simulink library "mbd_s32k1xx_ec_toolbox"  (Simulink 9.0)
settings: Solver=FixedStepDiscrete  StartTime=0.0  StopTime=10.0  FixedStep=0.1  RelTol=1e-3  EnableMultiTasking=on
InitFcn:
  | mbd_s32k_consistency_checks(bdroot(gcs));
(part 4 of 8)

== system mbd_s32k1xx_ec_toolbox/Core and System Blocks/DMA Blocks ==
  eDMA_Config : S-Function  FunctionName=edma_s32k_config  SFunctionDeploymentMode=off  EnableBusSupport=off  mask(edma_s32k_config){channel=0, show_advanced_tab=on, channel_advanced_checkbox=off, show_enabled=on, arbitration=EDMA_ARBITRATION_FIXED_PRIORITY, halt_on_error=false, channel0priority=EDMA_CHN_DEFAULT_PRIORITY, channel0requestsource=EDMA_REQ_DISABLED, channel0enable=off, channel1priority=EDMA_CHN_DEFAULT_PRIORITY, channel1requestsource=EDMA_REQ_DISABLED, channel1enable=off, channel2priority=EDMA_CHN_DEFAULT_PRIORITY, channel2requestsource=EDMA_REQ_DISABLED, channel2enable=off, channel3priority=EDMA_CHN_DEFAULT_PRIORITY, channel3requestsource=EDMA_REQ_DISABLED, channel3enable=off, channel4priority=EDMA_CHN_DEFAULT_PRIORITY, channel4requestsource=EDMA_REQ_DISABLED, channel4enable=off, channel5priority=EDMA_CHN_DEFAULT_PRIORITY, channel5requestsource=EDMA_REQ_DISABLED, channel5enable=off, channel6priority=EDMA_CHN_DEFAULT_PRIORITY, channel6requestsource=EDMA_REQ_DISABLED, channel6enable=off, channel7priority=EDMA_CHN_DEFAULT_PRIORITY, channel7requestsource=EDMA_REQ_DISABLED, channel7enable=off, channel8priority=EDMA_CHN_DEFAULT_PRIORITY, channel8requestsource=EDMA_REQ_DISABLED, channel8enable=off, channel9priority=EDMA_CHN_DEFAULT_PRIORITY, channel9requestsource=EDMA_REQ_DISABLED, channel9enable=off, channel10priority=EDMA_CHN_DEFAULT_PRIORITY, channel10requestsource=EDMA_REQ_DISABLED, channel10enable=off, channel11priority=EDMA_CHN_DEFAULT_PRIORITY, channel11requestsource=EDMA_REQ_DISABLED, channel11enable=off, channel12priority=EDMA_CHN_DEFAULT_PRIORITY, channel12requestsource=EDMA_REQ_DISABLED, channel12enable=off, channel13priority=EDMA_CHN_DEFAULT_PRIORITY, channel13requestsource=EDMA_REQ_DISABLED, channel13enable=off, channel14priority=EDMA_CHN_DEFAULT_PRIORITY, channel14requestsource=EDMA_REQ_DISABLED, channel14enable=off, channel15priority=EDMA_CHN_DEFAULT_PRIORITY, channel15requestsource=EDMA_REQ_DISABLED, channel15enable=off}
      mask prompts: show_advanced_tab "Show advanced global settings"; channel_advanced_checkbox "Show channel settings"; show_enabled "Show enabled channels"; halt_on_error "Halt on error"; channel0priority "Priority"; channel0requestsource "DMA request source"; channel0enable "Enable"; channel1priority "Priority"; channel1requestsource "DMA request source"; channel1enable "Enable"; channel2priority "Priority"; channel2requestsource "DMA request source"; channel2enable "Enable"; channel3priority "Priority"; channel3requestsource "DMA request source"; channel3enable "Enable"; channel4priority "Priority"; channel4requestsource "DMA request source"; channel4enable "Enable"; channel5priority "Priority"; channel5requestsource "DMA request source"; channel5enable "Enable"; channel6priority "Priority"; channel6requestsource "DMA request source"; channel6enable "Enable"; channel7priority "Priority"; channel7requestsource "DMA request source"; channel7enable "Enable"; channel8priority "Priority"; channel8requestsource "DMA request source"; channel8enable "Enable"; channel9priority "Priority"; channel9requestsource "DMA request source"; channel9enable "Enable"; channel10priority "Priority"; channel10requestsource "DMA request source"; channel10enable "Enable"; channel11priority "Priority"; channel11requestsource "DMA request source"; channel11enable "Enable"; channel12priority "Priority"; channel12requestsource "DMA request source"; channel12enable "Enable"; channel13priority "Priority"; channel13requestsource "DMA request source"; channel13enable "Enable"; channel14priority "Priority"; channel14requestsource "DMA request source"; channel14enable "Enable"; channel15priority "Priority"; channel15requestsource "DMA request source"; channel15enable "Enable"
      mask help: This block allows the user to configure the eDMA module and all of its channels.
      mask init:
      | maskStr = mbd_s32k_edma_config_init();
      settings: NameChangeFcn=mbd_s32k_name_check(gcb);
      mask Help: web(fullfile(mbd_s32k_block_help, 'edma', 'edma_config.html'));
      mask TypeOptions channel: 0 | 1 | 2 | 3 | 4 | 5 | 6 | 7 | 8 | 9 | 10 | 11 | 12 | 13 | 14 | 15
      mask Callback channel: mbd_s32k_edma_config_cbk()
      mask Callback show_advanced_tab: mbd_s32k_edma_config_cbk()
      mask Callback channel_advanced_checkbox: mbd_s32k_edma_config_cbk()
      mask Callback show_enabled: mbd_s32k_edma_config_en_chn()
      mask TypeOptions arbitration: EDMA_ARBITRATION_FIXED_PRIORITY | EDMA_ARBITRATION_ROUND_ROBIN
      mask TypeOptions halt_on_error: false | true
      mask TypeOptions channel0priority: EDMA_CHN_DEFAULT_PRIORITY | EDMA_CHN_PRIORITY_0 | EDMA_CHN_PRIORITY_1 | EDMA_CHN_PRIORITY_2 | EDMA_CHN_PRIORITY_3 | EDMA_CHN_PRIORITY_4 | EDMA_CHN_PRIORITY_5 | EDMA_CHN_PRIORITY_6 | EDMA_CHN_PRIORITY_7 | EDMA_CHN_PRIORITY_8 | EDMA_CHN_PRIORITY_9 | EDMA_CHN_PRIORITY_10 | EDMA_CHN_PRIORITY_11 | EDMA_CHN_PRIORITY_12 | EDMA_CHN_PRIORITY_13 | EDMA_CHN_PRIORITY_14 | EDMA_CHN_PRIORITY_15
      mask Callback channel0priority: mbd_s32k_edma_transfer_priority_cbk('0')
      mask TypeOptions channel0requestsource: EDMA_REQ_DISABLED | EDMA_REQ_LPUART0_RX | EDMA_REQ_LPUART0_TX | EDMA_REQ_LPUART1_RX | EDMA_REQ_LPUART1_TX | EDMA_REQ_FLEXIO_SHIFTER0 | EDMA_REQ_FLEXIO_SHIFTER1 | EDMA_REQ_FLEXIO_SHIFTER2 | EDMA_REQ_FLEXIO_SHIFTER3 | EDMA_REQ_LPSPI0_RX | EDMA_REQ_LPSPI0_TX | EDMA_REQ_LPSPI1_RX | EDMA_REQ_LPSPI1_TX | EDMA_REQ_FTM1_CHANNEL_0 | EDMA_REQ_FTM1_CHANNEL_1 | EDMA_REQ_FTM1_CHANNEL_2 | EDMA_REQ_FTM1_CHANNEL_3 | EDMA_REQ_FTM1_CHANNEL_4 | EDMA_REQ_FTM1_CHANNEL_5 | EDMA_REQ_FTM1_CHANNEL_6 | EDMA_REQ_FTM1_CHANNEL_7 | EDMA_REQ_FTM2_CHANNEL_0 | EDMA_REQ_FTM2_CHANNEL_1 | EDMA_REQ_FTM2_CHANNEL_2 | EDMA_REQ_FTM2_CHANNEL_3 | EDMA_REQ_FTM2_CHANNEL_4 | EDMA_REQ_FTM2_CHANNEL_5 | EDMA_REQ_FTM2_CHANNEL_6 | EDMA_REQ_FTM2_CHANNEL_7 | EDMA_REQ_FTM0_OR_CH0_CH7 | EDMA_REQ_FTM3_OR_CH0_CH7 | EDMA_REQ_ADC0 | EDMA_REQ_ADC1 | EDMA_REQ_LPI2C0_RX | EDMA_REQ_LPI2C0_TX | EDMA_REQ_PDB0 | EDMA_REQ_PDB1 | EDMA_REQ_CMP0 | EDMA_REQ_PORTA | EDMA_REQ_PORTB | EDMA_REQ_PORTC | EDMA_REQ_PORTD | EDMA_REQ_PORTE | EDMA_REQ_FLEXCAN0 | EDMA_REQ_FLEXCAN1 | EDMA_REQ_LPTMR0 | EDMA_REQ_DMAMUX_ALWAYS_ENABLED0 | EDMA_REQ_DMAMUX_ALWAYS_ENABLED1
      mask Callback channel0enable: mbd_s32k_edma_config_en_chn()
      mask TypeOptions channel1priority: EDMA_CHN_DEFAULT_PRIORITY | EDMA_CHN_PRIORITY_0 | EDMA_CHN_PRIORITY_1 | EDMA_CHN_PRIORITY_2 | EDMA_CHN_PRIORITY_3 | EDMA_CHN_PRIORITY_4 | EDMA_CHN_PRIORITY_5 | EDMA_CHN_PRIORITY_6 | EDMA_CHN_PRIORITY_7 | EDMA_CHN_PRIORITY_8 | EDMA_CHN_PRIORITY_9 | EDMA_CHN_PRIORITY_10 | EDMA_CHN_PRIORITY_11 | EDMA_CHN_PRIORITY_12 | EDMA_CHN_PRIORITY_13 | EDMA_CHN_PRIORITY_14 | EDMA_CHN_PRIORITY_15
      mask Callback channel1priority: mbd_s32k_edma_transfer_priority_cbk('1')
      mask TypeOptions channel1requestsource: EDMA_REQ_DISABLED | EDMA_REQ_LPUART0_RX | EDMA_REQ_LPUART0_TX | EDMA_REQ_LPUART1_RX | EDMA_REQ_LPUART1_TX | EDMA_REQ_FLEXIO_SHIFTER0 | EDMA_REQ_FLEXIO_SHIFTER1 | EDMA_REQ_FLEXIO_SHIFTER2 | EDMA_REQ_FLEXIO_SHIFTER3 | EDMA_REQ_LPSPI0_RX | EDMA_REQ_LPSPI0_TX | EDMA_REQ_LPSPI1_RX | EDMA_REQ_LPSPI1_TX | EDMA_REQ_FTM1_CHANNEL_0 | EDMA_REQ_FTM1_CHANNEL_1 | EDMA_REQ_FTM1_CHANNEL_2 | EDMA_REQ_FTM1_CHANNEL_3 | EDMA_REQ_FTM1_CHANNEL_4 | EDMA_REQ_FTM1_CHANNEL_5 | EDMA_REQ_FTM1_CHANNEL_6 | EDMA_REQ_FTM1_CHANNEL_7 | EDMA_REQ_FTM2_CHANNEL_0 | EDMA_REQ_FTM2_CHANNEL_1 | EDMA_REQ_FTM2_CHANNEL_2 | EDMA_REQ_FTM2_CHANNEL_3 | EDMA_REQ_FTM2_CHANNEL_4 | EDMA_REQ_FTM2_CHANNEL_5 | EDMA_REQ_FTM2_CHANNEL_6 | EDMA_REQ_FTM2_CHANNEL_7 | EDMA_REQ_FTM0_OR_CH0_CH7 | EDMA_REQ_FTM3_OR_CH0_CH7 | EDMA_REQ_ADC0 | EDMA_REQ_ADC1 | EDMA_REQ_LPI2C0_RX | EDMA_REQ_LPI2C0_TX | EDMA_REQ_PDB0 | EDMA_REQ_PDB1 | EDMA_REQ_CMP0 | EDMA_REQ_PORTA | EDMA_REQ_PORTB | EDMA_REQ_PORTC | EDMA_REQ_PORTD | EDMA_REQ_PORTE | EDMA_REQ_FLEXCAN0 | EDMA_REQ_FLEXCAN1 | EDMA_REQ_LPTMR0 | EDMA_REQ_DMAMUX_ALWAYS_ENABLED0 | EDMA_REQ_DMAMUX_ALWAYS_ENABLED1
      mask Callback channel1enable: mbd_s32k_edma_config_en_chn()
      mask TypeOptions channel2priority: EDMA_CHN_DEFAULT_PRIORITY | EDMA_CHN_PRIORITY_0 | EDMA_CHN_PRIORITY_1 | EDMA_CHN_PRIORITY_2 | EDMA_CHN_PRIORITY_3 | EDMA_CHN_PRIORITY_4 | EDMA_CHN_PRIORITY_5 | EDMA_CHN_PRIORITY_6 | EDMA_CHN_PRIORITY_7 | EDMA_CHN_PRIORITY_8 | EDMA_CHN_PRIORITY_9 | EDMA_CHN_PRIORITY_10 | EDMA_CHN_PRIORITY_11 | EDMA_CHN_PRIORITY_12 | EDMA_CHN_PRIORITY_13 | EDMA_CHN_PRIORITY_14 | EDMA_CHN_PRIORITY_15
      mask Callback channel2priority: mbd_s32k_edma_transfer_priority_cbk('2')
      mask TypeOptions channel2requestsource: EDMA_REQ_DISABLED | EDMA_REQ_LPUART0_RX | EDMA_REQ_LPUART0_TX | EDMA_REQ_LPUART1_RX | EDMA_REQ_LPUART1_TX | EDMA_REQ_FLEXIO_SHIFTER0 | EDMA_REQ_FLEXIO_SHIFTER1 | EDMA_REQ_FLEXIO_SHIFTER2 | EDMA_REQ_FLEXIO_SHIFTER3 | EDMA_REQ_LPSPI0_RX | EDMA_REQ_LPSPI0_TX | EDMA_REQ_LPSPI1_RX | EDMA_REQ_LPSPI1_TX | EDMA_REQ_FTM1_CHANNEL_0 | EDMA_REQ_FTM1_CHANNEL_1 | EDMA_REQ_FTM1_CHANNEL_2 | EDMA_REQ_FTM1_CHANNEL_3 | EDMA_REQ_FTM1_CHANNEL_4 | EDMA_REQ_FTM1_CHANNEL_5 | EDMA_REQ_FTM1_CHANNEL_6 | EDMA_REQ_FTM1_CHANNEL_7 | EDMA_REQ_FTM2_CHANNEL_0 | EDMA_REQ_FTM2_CHANNEL_1 | EDMA_REQ_FTM2_CHANNEL_2 | EDMA_REQ_FTM2_CHANNEL_3 | EDMA_REQ_FTM2_CHANNEL_4 | EDMA_REQ_FTM2_CHANNEL_5 | EDMA_REQ_FTM2_CHANNEL_6 | EDMA_REQ_FTM2_CHANNEL_7 | EDMA_REQ_FTM0_OR_CH0_CH7 | EDMA_REQ_FTM3_OR_CH0_CH7 | EDMA_REQ_ADC0 | EDMA_REQ_ADC1 | EDMA_REQ_LPI2C0_RX | EDMA_REQ_LPI2C0_TX | EDMA_REQ_PDB0 | EDMA_REQ_PDB1 | EDMA_REQ_CMP0 | EDMA_REQ_PORTA | EDMA_REQ_PORTB | EDMA_REQ_PORTC | EDMA_REQ_PORTD | EDMA_REQ_PORTE | EDMA_REQ_FLEXCAN0 | EDMA_REQ_FLEXCAN1 | EDMA_REQ_LPTMR0 | EDMA_REQ_DMAMUX_ALWAYS_ENABLED0 | EDMA_REQ_DMAMUX_ALWAYS_ENABLED1
      mask Callback channel2enable: mbd_s32k_edma_config_en_chn()
      mask TypeOptions channel3priority: EDMA_CHN_DEFAULT_PRIORITY | EDMA_CHN_PRIORITY_0 | EDMA_CHN_PRIORITY_1 | EDMA_CHN_PRIORITY_2 | EDMA_CHN_PRIORITY_3 | EDMA_CHN_PRIORITY_4 | EDMA_CHN_PRIORITY_5 | EDMA_CHN_PRIORITY_6 | EDMA_CHN_PRIORITY_7 | EDMA_CHN_PRIORITY_8 | EDMA_CHN_PRIORITY_9 | EDMA_CHN_PRIORITY_10 | EDMA_CHN_PRIORITY_11 | EDMA_CHN_PRIORITY_12 | EDMA_CHN_PRIORITY_13 | EDMA_CHN_PRIORITY_14 | EDMA_CHN_PRIORITY_15
      mask Callback channel3priority: mbd_s32k_edma_transfer_priority_cbk('3')
      mask TypeOptions channel3requestsource: EDMA_REQ_DISABLED | EDMA_REQ_LPUART0_RX | EDMA_REQ_LPUART0_TX | EDMA_REQ_LPUART1_RX | EDMA_REQ_LPUART1_TX | EDMA_REQ_FLEXIO_SHIFTER0 | EDMA_REQ_FLEXIO_SHIFTER1 | EDMA_REQ_FLEXIO_SHIFTER2 | EDMA_REQ_FLEXIO_SHIFTER3 | EDMA_REQ_LPSPI0_RX | EDMA_REQ_LPSPI0_TX | EDMA_REQ_LPSPI1_RX | EDMA_REQ_LPSPI1_TX | EDMA_REQ_FTM1_CHANNEL_0 | EDMA_REQ_FTM1_CHANNEL_1 | EDMA_REQ_FTM1_CHANNEL_2 | EDMA_REQ_FTM1_CHANNEL_3 | EDMA_REQ_FTM1_CHANNEL_4 | EDMA_REQ_FTM1_CHANNEL_5 | EDMA_REQ_FTM1_CHANNEL_6 | EDMA_REQ_FTM1_CHANNEL_7 | EDMA_REQ_FTM2_CHANNEL_0 | EDMA_REQ_FTM2_CHANNEL_1 | EDMA_REQ_FTM2_CHANNEL_2 | EDMA_REQ_FTM2_CHANNEL_3 | EDMA_REQ_FTM2_CHANNEL_4 | EDMA_REQ_FTM2_CHANNEL_5 | EDMA_REQ_FTM2_CHANNEL_6 | EDMA_REQ_FTM2_CHANNEL_7 | EDMA_REQ_FTM0_OR_CH0_CH7 | EDMA_REQ_FTM3_OR_CH0_CH7 | EDMA_REQ_ADC0 | EDMA_REQ_ADC1 | EDMA_REQ_LPI2C0_RX | EDMA_REQ_LPI2C0_TX | EDMA_REQ_PDB0 | EDMA_REQ_PDB1 | EDMA_REQ_CMP0 | EDMA_REQ_PORTA | EDMA_REQ_PORTB | EDMA_REQ_PORTC | EDMA_REQ_PORTD | EDMA_REQ_PORTE | EDMA_REQ_FLEXCAN0 | EDMA_REQ_FLEXCAN1 | EDMA_REQ_LPTMR0 | EDMA_REQ_DMAMUX_ALWAYS_ENABLED0 | EDMA_REQ_DMAMUX_ALWAYS_ENABLED1
      mask Callback channel3enable: mbd_s32k_edma_config_en_chn()
      mask TypeOptions channel4priority: EDMA_CHN_DEFAULT_PRIORITY | EDMA_CHN_PRIORITY_0 | EDMA_CHN_PRIORITY_1 | EDMA_CHN_PRIORITY_2 | EDMA_CHN_PRIORITY_3 | EDMA_CHN_PRIORITY_4 | EDMA_CHN_PRIORITY_5 | EDMA_CHN_PRIORITY_6 | EDMA_CHN_PRIORITY_7 | EDMA_CHN_PRIORITY_8 | EDMA_CHN_PRIORITY_9 | EDMA_CHN_PRIORITY_10 | EDMA_CHN_PRIORITY_11 | EDMA_CHN_PRIORITY_12 | EDMA_CHN_PRIORITY_13 | EDMA_CHN_PRIORITY_14 | EDMA_CHN_PRIORITY_15
      mask Callback channel4priority: mbd_s32k_edma_transfer_priority_cbk('4')
      mask TypeOptions channel4requestsource: EDMA_REQ_DISABLED | EDMA_REQ_LPUART0_RX | EDMA_REQ_LPUART0_TX | EDMA_REQ_LPUART1_RX | EDMA_REQ_LPUART1_TX | EDMA_REQ_FLEXIO_SHIFTER0 | EDMA_REQ_FLEXIO_SHIFTER1 | EDMA_REQ_FLEXIO_SHIFTER2 | EDMA_REQ_FLEXIO_SHIFTER3 | EDMA_REQ_LPSPI0_RX | EDMA_REQ_LPSPI0_TX | EDMA_REQ_LPSPI1_RX | EDMA_REQ_LPSPI1_TX | EDMA_REQ_FTM1_CHANNEL_0 | EDMA_REQ_FTM1_CHANNEL_1 | EDMA_REQ_FTM1_CHANNEL_2 | EDMA_REQ_FTM1_CHANNEL_3 | EDMA_REQ_FTM1_CHANNEL_4 | EDMA_REQ_FTM1_CHANNEL_5 | EDMA_REQ_FTM1_CHANNEL_6 | EDMA_REQ_FTM1_CHANNEL_7 | EDMA_REQ_FTM2_CHANNEL_0 | EDMA_REQ_FTM2_CHANNEL_1 | EDMA_REQ_FTM2_CHANNEL_2 | EDMA_REQ_FTM2_CHANNEL_3 | EDMA_REQ_FTM2_CHANNEL_4 | EDMA_REQ_FTM2_CHANNEL_5 | EDMA_REQ_FTM2_CHANNEL_6 | EDMA_REQ_FTM2_CHANNEL_7 | EDMA_REQ_FTM0_OR_CH0_CH7 | EDMA_REQ_FTM3_OR_CH0_CH7 | EDMA_REQ_ADC0 | EDMA_REQ_ADC1 | EDMA_REQ_LPI2C0_RX | EDMA_REQ_LPI2C0_TX | EDMA_REQ_PDB0 | EDMA_REQ_PDB1 | EDMA_REQ_CMP0 | EDMA_REQ_PORTA | EDMA_REQ_PORTB | EDMA_REQ_PORTC | EDMA_REQ_PORTD | EDMA_REQ_PORTE | EDMA_REQ_FLEXCAN0 | EDMA_REQ_FLEXCAN1 | EDMA_REQ_LPTMR0 | EDMA_REQ_DMAMUX_ALWAYS_ENABLED0 | EDMA_REQ_DMAMUX_ALWAYS_ENABLED1
      mask Callback channel4enable: mbd_s32k_edma_config_en_chn()
      mask TypeOptions channel5priority: EDMA_CHN_DEFAULT_PRIORITY | EDMA_CHN_PRIORITY_0 | EDMA_CHN_PRIORITY_1 | EDMA_CHN_PRIORITY_2 | EDMA_CHN_PRIORITY_3 | EDMA_CHN_PRIORITY_4 | EDMA_CHN_PRIORITY_5 | EDMA_CHN_PRIORITY_6 | EDMA_CHN_PRIORITY_7 | EDMA_CHN_PRIORITY_8 | EDMA_CHN_PRIORITY_9 | EDMA_CHN_PRIORITY_10 | EDMA_CHN_PRIORITY_11 | EDMA_CHN_PRIORITY_12 | EDMA_CHN_PRIORITY_13 | EDMA_CHN_PRIORITY_14 | EDMA_CHN_PRIORITY_15
      mask Callback channel5priority: mbd_s32k_edma_transfer_priority_cbk('5')
      mask TypeOptions channel5requestsource: EDMA_REQ_DISABLED | EDMA_REQ_LPUART0_RX | EDMA_REQ_LPUART0_TX | EDMA_REQ_LPUART1_RX | EDMA_REQ_LPUART1_TX | EDMA_REQ_FLEXIO_SHIFTER0 | EDMA_REQ_FLEXIO_SHIFTER1 | EDMA_REQ_FLEXIO_SHIFTER2 | EDMA_REQ_FLEXIO_SHIFTER3 | EDMA_REQ_LPSPI0_RX | EDMA_REQ_LPSPI0_TX | EDMA_REQ_LPSPI1_RX | EDMA_REQ_LPSPI1_TX | EDMA_REQ_FTM1_CHANNEL_0 | EDMA_REQ_FTM1_CHANNEL_1 | EDMA_REQ_FTM1_CHANNEL_2 | EDMA_REQ_FTM1_CHANNEL_3 | EDMA_REQ_FTM1_CHANNEL_4 | EDMA_REQ_FTM1_CHANNEL_5 | EDMA_REQ_FTM1_CHANNEL_6 | EDMA_REQ_FTM1_CHANNEL_7 | EDMA_REQ_FTM2_CHANNEL_0 | EDMA_REQ_FTM2_CHANNEL_1 | EDMA_REQ_FTM2_CHANNEL_2 | EDMA_REQ_FTM2_CHANNEL_3 | EDMA_REQ_FTM2_CHANNEL_4 | EDMA_REQ_FTM2_CHANNEL_5 | EDMA_REQ_FTM2_CHANNEL_6 | EDMA_REQ_FTM2_CHANNEL_7 | EDMA_REQ_FTM0_OR_CH0_CH7 | EDMA_REQ_FTM3_OR_CH0_CH7 | EDMA_REQ_ADC0 | EDMA_REQ_ADC1 | EDMA_REQ_LPI2C0_RX | EDMA_REQ_LPI2C0_TX | EDMA_REQ_PDB0 | EDMA_REQ_PDB1 | EDMA_REQ_CMP0 | EDMA_REQ_PORTA | EDMA_REQ_PORTB | EDMA_REQ_PORTC | EDMA_REQ_PORTD | EDMA_REQ_PORTE | EDMA_REQ_FLEXCAN0 | EDMA_REQ_FLEXCAN1 | EDMA_REQ_LPTMR0 | EDMA_REQ_DMAMUX_ALWAYS_ENABLED0 | EDMA_REQ_DMAMUX_ALWAYS_ENABLED1
      mask Callback channel5enable: mbd_s32k_edma_config_en_chn()
      mask TypeOptions channel6priority: EDMA_CHN_DEFAULT_PRIORITY | EDMA_CHN_PRIORITY_0 | EDMA_CHN_PRIORITY_1 | EDMA_CHN_PRIORITY_2 | EDMA_CHN_PRIORITY_3 | EDMA_CHN_PRIORITY_4 | EDMA_CHN_PRIORITY_5 | EDMA_CHN_PRIORITY_6 | EDMA_CHN_PRIORITY_7 | EDMA_CHN_PRIORITY_8 | EDMA_CHN_PRIORITY_9 | EDMA_CHN_PRIORITY_10 | EDMA_CHN_PRIORITY_11 | EDMA_CHN_PRIORITY_12 | EDMA_CHN_PRIORITY_13 | EDMA_CHN_PRIORITY_14 | EDMA_CHN_PRIORITY_15
      mask Callback channel6priority: mbd_s32k_edma_transfer_priority_cbk('6')
      mask TypeOptions channel6requestsource: EDMA_REQ_DISABLED | EDMA_REQ_LPUART0_RX | EDMA_REQ_LPUART0_TX | EDMA_REQ_LPUART1_RX | EDMA_REQ_LPUART1_TX | EDMA_REQ_FLEXIO_SHIFTER0 | EDMA_REQ_FLEXIO_SHIFTER1 | EDMA_REQ_FLEXIO_SHIFTER2 | EDMA_REQ_FLEXIO_SHIFTER3 | EDMA_REQ_LPSPI0_RX | EDMA_REQ_LPSPI0_TX | EDMA_REQ_LPSPI1_RX | EDMA_REQ_LPSPI1_TX | EDMA_REQ_FTM1_CHANNEL_0 | EDMA_REQ_FTM1_CHANNEL_1 | EDMA_REQ_FTM1_CHANNEL_2 | EDMA_REQ_FTM1_CHANNEL_3 | EDMA_REQ_FTM1_CHANNEL_4 | EDMA_REQ_FTM1_CHANNEL_5 | EDMA_REQ_FTM1_CHANNEL_6 | EDMA_REQ_FTM1_CHANNEL_7 | EDMA_REQ_FTM2_CHANNEL_0 | EDMA_REQ_FTM2_CHANNEL_1 | EDMA_REQ_FTM2_CHANNEL_2 | EDMA_REQ_FTM2_CHANNEL_3 | EDMA_REQ_FTM2_CHANNEL_4 | EDMA_REQ_FTM2_CHANNEL_5 | EDMA_REQ_FTM2_CHANNEL_6 | EDMA_REQ_FTM2_CHANNEL_7 | EDMA_REQ_FTM0_OR_CH0_CH7 | EDMA_REQ_FTM3_OR_CH0_CH7 | EDMA_REQ_ADC0 | EDMA_REQ_ADC1 | EDMA_REQ_LPI2C0_RX | EDMA_REQ_LPI2C0_TX | EDMA_REQ_PDB0 | EDMA_REQ_PDB1 | EDMA_REQ_CMP0 | EDMA_REQ_PORTA | EDMA_REQ_PORTB | EDMA_REQ_PORTC | EDMA_REQ_PORTD | EDMA_REQ_PORTE | EDMA_REQ_FLEXCAN0 | EDMA_REQ_FLEXCAN1 | EDMA_REQ_LPTMR0 | EDMA_REQ_DMAMUX_ALWAYS_ENABLED0 | EDMA_REQ_DMAMUX_ALWAYS_ENABLED1
      mask Callback channel6enable: mbd_s32k_edma_config_en_chn()
      mask TypeOptions channel7priority: EDMA_CHN_DEFAULT_PRIORITY | EDMA_CHN_PRIORITY_0 | EDMA_CHN_PRIORITY_1 | EDMA_CHN_PRIORITY_2 | EDMA_CHN_PRIORITY_3 | EDMA_CHN_PRIORITY_4 | EDMA_CHN_PRIORITY_5 | EDMA_CHN_PRIORITY_6 | EDMA_CHN_PRIORITY_7 | EDMA_CHN_PRIORITY_8 | EDMA_CHN_PRIORITY_9 | EDMA_CHN_PRIORITY_10 | EDMA_CHN_PRIORITY_11 | EDMA_CHN_PRIORITY_12 | EDMA_CHN_PRIORITY_13 | EDMA_CHN_PRIORITY_14 | EDMA_CHN_PRIORITY_15
      mask Callback channel7priority: mbd_s32k_edma_transfer_priority_cbk('7')
      mask TypeOptions channel7requestsource: EDMA_REQ_DISABLED | EDMA_REQ_LPUART0_RX | EDMA_REQ_LPUART0_TX | EDMA_REQ_LPUART1_RX | EDMA_REQ_LPUART1_TX | EDMA_REQ_FLEXIO_SHIFTER0 | EDMA_REQ_FLEXIO_SHIFTER1 | EDMA_REQ_FLEXIO_SHIFTER2 | EDMA_REQ_FLEXIO_SHIFTER3 | EDMA_REQ_LPSPI0_RX | EDMA_REQ_LPSPI0_TX | EDMA_REQ_LPSPI1_RX | EDMA_REQ_LPSPI1_TX | EDMA_REQ_FTM1_CHANNEL_0 | EDMA_REQ_FTM1_CHANNEL_1 | EDMA_REQ_FTM1_CHANNEL_2 | EDMA_REQ_FTM1_CHANNEL_3 | EDMA_REQ_FTM1_CHANNEL_4 | EDMA_REQ_FTM1_CHANNEL_5 | EDMA_REQ_FTM1_CHANNEL_6 | EDMA_REQ_FTM1_CHANNEL_7 | EDMA_REQ_FTM2_CHANNEL_0 | EDMA_REQ_FTM2_CHANNEL_1 | EDMA_REQ_FTM2_CHANNEL_2 | EDMA_REQ_FTM2_CHANNEL_3 | EDMA_REQ_FTM2_CHANNEL_4 | EDMA_REQ_FTM2_CHANNEL_5 | EDMA_REQ_FTM2_CHANNEL_6 | EDMA_REQ_FTM2_CHANNEL_7 | EDMA_REQ_FTM0_OR_CH0_CH7 | EDMA_REQ_FTM3_OR_CH0_CH7 | EDMA_REQ_ADC0 | EDMA_REQ_ADC1 | EDMA_REQ_LPI2C0_RX | EDMA_REQ_LPI2C0_TX | EDMA_REQ_PDB0 | EDMA_REQ_PDB1 | EDMA_REQ_CMP0 | EDMA_REQ_PORTA | EDMA_REQ_PORTB | EDMA_REQ_PORTC | EDMA_REQ_PORTD | EDMA_REQ_PORTE | EDMA_REQ_FLEXCAN0 | EDMA_REQ_FLEXCAN1 | EDMA_REQ_LPTMR0 | EDMA_REQ_DMAMUX_ALWAYS_ENABLED0 | EDMA_REQ_DMAMUX_ALWAYS_ENABLED1
      mask Callback channel7enable: mbd_s32k_edma_config_en_chn()
      mask TypeOptions channel8priority: EDMA_CHN_DEFAULT_PRIORITY | EDMA_CHN_PRIORITY_0 | EDMA_CHN_PRIORITY_1 | EDMA_CHN_PRIORITY_2 | EDMA_CHN_PRIORITY_3 | EDMA_CHN_PRIORITY_4 | EDMA_CHN_PRIORITY_5 | EDMA_CHN_PRIORITY_6 | EDMA_CHN_PRIORITY_7 | EDMA_CHN_PRIORITY_8 | EDMA_CHN_PRIORITY_9 | EDMA_CHN_PRIORITY_10 | EDMA_CHN_PRIORITY_11 | EDMA_CHN_PRIORITY_12 | EDMA_CHN_PRIORITY_13 | EDMA_CHN_PRIORITY_14 | EDMA_CHN_PRIORITY_15
      mask Callback channel8priority: mbd_s32k_edma_transfer_priority_cbk('8')
      mask TypeOptions channel8requestsource: EDMA_REQ_DISABLED | EDMA_REQ_LPUART0_RX | EDMA_REQ_LPUART0_TX | EDMA_REQ_LPUART1_RX | EDMA_REQ_LPUART1_TX | EDMA_REQ_FLEXIO_SHIFTER0 | EDMA_REQ_FLEXIO_SHIFTER1 | EDMA_REQ_FLEXIO_SHIFTER2 | EDMA_REQ_FLEXIO_SHIFTER3 | EDMA_REQ_LPSPI0_RX | EDMA_REQ_LPSPI0_TX | EDMA_REQ_LPSPI1_RX | EDMA_REQ_LPSPI1_TX | EDMA_REQ_FTM1_CHANNEL_0 | EDMA_REQ_FTM1_CHANNEL_1 | EDMA_REQ_FTM1_CHANNEL_2 | EDMA_REQ_FTM1_CHANNEL_3 | EDMA_REQ_FTM1_CHANNEL_4 | EDMA_REQ_FTM1_CHANNEL_5 | EDMA_REQ_FTM1_CHANNEL_6 | EDMA_REQ_FTM1_CHANNEL_7 | EDMA_REQ_FTM2_CHANNEL_0 | EDMA_REQ_FTM2_CHANNEL_1 | EDMA_REQ_FTM2_CHANNEL_2 | EDMA_REQ_FTM2_CHANNEL_3 | EDMA_REQ_FTM2_CHANNEL_4 | EDMA_REQ_FTM2_CHANNEL_5 | EDMA_REQ_FTM2_CHANNEL_6 | EDMA_REQ_FTM2_CHANNEL_7 | EDMA_REQ_FTM0_OR_CH0_CH7 | EDMA_REQ_FTM3_OR_CH0_CH7 | EDMA_REQ_ADC0 | EDMA_REQ_ADC1 | EDMA_REQ_LPI2C0_RX | EDMA_REQ_LPI2C0_TX | EDMA_REQ_PDB0 | EDMA_REQ_PDB1 | EDMA_REQ_CMP0 | EDMA_REQ_PORTA | EDMA_REQ_PORTB | EDMA_REQ_PORTC | EDMA_REQ_PORTD | EDMA_REQ_PORTE | EDMA_REQ_FLEXCAN0 | EDMA_REQ_FLEXCAN1 | EDMA_REQ_LPTMR0 | EDMA_REQ_DMAMUX_ALWAYS_ENABLED0 | EDMA_REQ_DMAMUX_ALWAYS_ENABLED1
      mask Callback channel8enable: mbd_s32k_edma_config_en_chn()
      mask TypeOptions channel9priority: EDMA_CHN_DEFAULT_PRIORITY | EDMA_CHN_PRIORITY_0 | EDMA_CHN_PRIORITY_1 | EDMA_CHN_PRIORITY_2 | EDMA_CHN_PRIORITY_3 | EDMA_CHN_PRIORITY_4 | EDMA_CHN_PRIORITY_5 | EDMA_CHN_PRIORITY_6 | EDMA_CHN_PRIORITY_7 | EDMA_CHN_PRIORITY_8 | EDMA_CHN_PRIORITY_9 | EDMA_CHN_PRIORITY_10 | EDMA_CHN_PRIORITY_11 | EDMA_CHN_PRIORITY_12 | EDMA_CHN_PRIORITY_13 | EDMA_CHN_PRIORITY_14 | EDMA_CHN_PRIORITY_15
      mask Callback channel9priority: mbd_s32k_edma_transfer_priority_cbk('9')
      mask TypeOptions channel9requestsource: EDMA_REQ_DISABLED | EDMA_REQ_LPUART0_RX | EDMA_REQ_LPUART0_TX | EDMA_REQ_LPUART1_RX | EDMA_REQ_LPUART1_TX | EDMA_REQ_FLEXIO_SHIFTER0 | EDMA_REQ_FLEXIO_SHIFTER1 | EDMA_REQ_FLEXIO_SHIFTER2 | EDMA_REQ_FLEXIO_SHIFTER3 | EDMA_REQ_LPSPI0_RX | EDMA_REQ_LPSPI0_TX | EDMA_REQ_LPSPI1_RX | EDMA_REQ_LPSPI1_TX | EDMA_REQ_FTM1_CHANNEL_0 | EDMA_REQ_FTM1_CHANNEL_1 | EDMA_REQ_FTM1_CHANNEL_2 | EDMA_REQ_FTM1_CHANNEL_3 | EDMA_REQ_FTM1_CHANNEL_4 | EDMA_REQ_FTM1_CHANNEL_5 | EDMA_REQ_FTM1_CHANNEL_6 | EDMA_REQ_FTM1_CHANNEL_7 | EDMA_REQ_FTM2_CHANNEL_0 | EDMA_REQ_FTM2_CHANNEL_1 | EDMA_REQ_FTM2_CHANNEL_2 | EDMA_REQ_FTM2_CHANNEL_3 | EDMA_REQ_FTM2_CHANNEL_4 | EDMA_REQ_FTM2_CHANNEL_5 | EDMA_REQ_FTM2_CHANNEL_6 | EDMA_REQ_FTM2_CHANNEL_7 | EDMA_REQ_FTM0_OR_CH0_CH7 | EDMA_REQ_FTM3_OR_CH0_CH7 | EDMA_REQ_ADC0 | EDMA_REQ_ADC1 | EDMA_REQ_LPI2C0_RX | EDMA_REQ_LPI2C0_TX | EDMA_REQ_PDB0 | EDMA_REQ_PDB1 | EDMA_REQ_CMP0 | EDMA_REQ_PORTA | EDMA_REQ_PORTB | EDMA_REQ_PORTC | EDMA_REQ_PORTD | EDMA_REQ_PORTE | EDMA_REQ_FLEXCAN0 | EDMA_REQ_FLEXCAN1 | EDMA_REQ_LPTMR0 | EDMA_REQ_DMAMUX_ALWAYS_ENABLED0 | EDMA_REQ_DMAMUX_ALWAYS_ENABLED1
      mask Callback channel9enable: mbd_s32k_edma_config_en_chn()
      mask TypeOptions channel10priority: EDMA_CHN_DEFAULT_PRIORITY | EDMA_CHN_PRIORITY_0 | EDMA_CHN_PRIORITY_1 | EDMA_CHN_PRIORITY_2 | EDMA_CHN_PRIORITY_3 | EDMA_CHN_PRIORITY_4 | EDMA_CHN_PRIORITY_5 | EDMA_CHN_PRIORITY_6 | EDMA_CHN_PRIORITY_7 | EDMA_CHN_PRIORITY_8 | EDMA_CHN_PRIORITY_9 | EDMA_CHN_PRIORITY_10 | EDMA_CHN_PRIORITY_11 | EDMA_CHN_PRIORITY_12 | EDMA_CHN_PRIORITY_13 | EDMA_CHN_PRIORITY_14 | EDMA_CHN_PRIORITY_15
      mask Callback channel10priority: mbd_s32k_edma_transfer_priority_cbk('10')
      mask TypeOptions channel10requestsource: EDMA_REQ_DISABLED | EDMA_REQ_LPUART0_RX | EDMA_REQ_LPUART0_TX | EDMA_REQ_LPUART1_RX | EDMA_REQ_LPUART1_TX | EDMA_REQ_FLEXIO_SHIFTER0 | EDMA_REQ_FLEXIO_SHIFTER1 | EDMA_REQ_FLEXIO_SHIFTER2 | EDMA_REQ_FLEXIO_SHIFTER3 | EDMA_REQ_LPSPI0_RX | EDMA_REQ_LPSPI0_TX | EDMA_REQ_LPSPI1_RX | EDMA_REQ_LPSPI1_TX | EDMA_REQ_FTM1_CHANNEL_0 | EDMA_REQ_FTM1_CHANNEL_1 | EDMA_REQ_FTM1_CHANNEL_2 | EDMA_REQ_FTM1_CHANNEL_3 | EDMA_REQ_FTM1_CHANNEL_4 | EDMA_REQ_FTM1_CHANNEL_5 | EDMA_REQ_FTM1_CHANNEL_6 | EDMA_REQ_FTM1_CHANNEL_7 | EDMA_REQ_FTM2_CHANNEL_0 | EDMA_REQ_FTM2_CHANNEL_1 | EDMA_REQ_FTM2_CHANNEL_2 | EDMA_REQ_FTM2_CHANNEL_3 | EDMA_REQ_FTM2_CHANNEL_4 | EDMA_REQ_FTM2_CHANNEL_5 | EDMA_REQ_FTM2_CHANNEL_6 | EDMA_REQ_FTM2_CHANNEL_7 | EDMA_REQ_FTM0_OR_CH0_CH7 | EDMA_REQ_FTM3_OR_CH0_CH7 | EDMA_REQ_ADC0 | EDMA_REQ_ADC1 | EDMA_REQ_LPI2C0_RX | EDMA_REQ_LPI2C0_TX | EDMA_REQ_PDB0 | EDMA_REQ_PDB1 | EDMA_REQ_CMP0 | EDMA_REQ_PORTA | EDMA_REQ_PORTB | EDMA_REQ_PORTC | EDMA_REQ_PORTD | EDMA_REQ_PORTE | EDMA_REQ_FLEXCAN0 | EDMA_REQ_FLEXCAN1 | EDMA_REQ_LPTMR0 | EDMA_REQ_DMAMUX_ALWAYS_ENABLED0 | EDMA_REQ_DMAMUX_ALWAYS_ENABLED1
      mask Callback channel10enable: mbd_s32k_edma_config_en_chn()
      mask TypeOptions channel11priority: EDMA_CHN_DEFAULT_PRIORITY | EDMA_CHN_PRIORITY_0 | EDMA_CHN_PRIORITY_1 | EDMA_CHN_PRIORITY_2 | EDMA_CHN_PRIORITY_3 | EDMA_CHN_PRIORITY_4 | EDMA_CHN_PRIORITY_5 | EDMA_CHN_PRIORITY_6 | EDMA_CHN_PRIORITY_7 | EDMA_CHN_PRIORITY_8 | EDMA_CHN_PRIORITY_9 | EDMA_CHN_PRIORITY_10 | EDMA_CHN_PRIORITY_11 | EDMA_CHN_PRIORITY_12 | EDMA_CHN_PRIORITY_13 | EDMA_CHN_PRIORITY_14 | EDMA_CHN_PRIORITY_15
      mask Callback channel11priority: mbd_s32k_edma_transfer_priority_cbk('11')
      mask TypeOptions channel11requestsource: EDMA_REQ_DISABLED | EDMA_REQ_LPUART0_RX | EDMA_REQ_LPUART0_TX | EDMA_REQ_LPUART1_RX | EDMA_REQ_LPUART1_TX | EDMA_REQ_FLEXIO_SHIFTER0 | EDMA_REQ_FLEXIO_SHIFTER1 | EDMA_REQ_FLEXIO_SHIFTER2 | EDMA_REQ_FLEXIO_SHIFTER3 | EDMA_REQ_LPSPI0_RX | EDMA_REQ_LPSPI0_TX | EDMA_REQ_LPSPI1_RX | EDMA_REQ_LPSPI1_TX | EDMA_REQ_FTM1_CHANNEL_0 | EDMA_REQ_FTM1_CHANNEL_1 | EDMA_REQ_FTM1_CHANNEL_2 | EDMA_REQ_FTM1_CHANNEL_3 | EDMA_REQ_FTM1_CHANNEL_4 | EDMA_REQ_FTM1_CHANNEL_5 | EDMA_REQ_FTM1_CHANNEL_6 | EDMA_REQ_FTM1_CHANNEL_7 | EDMA_REQ_FTM2_CHANNEL_0 | EDMA_REQ_FTM2_CHANNEL_1 | EDMA_REQ_FTM2_CHANNEL_2 | EDMA_REQ_FTM2_CHANNEL_3 | EDMA_REQ_FTM2_CHANNEL_4 | EDMA_REQ_FTM2_CHANNEL_5 | EDMA_REQ_FTM2_CHANNEL_6 | EDMA_REQ_FTM2_CHANNEL_7 | EDMA_REQ_FTM0_OR_CH0_CH7 | EDMA_REQ_FTM3_OR_CH0_CH7 | EDMA_REQ_ADC0 | EDMA_REQ_ADC1 | EDMA_REQ_LPI2C0_RX | EDMA_REQ_LPI2C0_TX | EDMA_REQ_PDB0 | EDMA_REQ_PDB1 | EDMA_REQ_CMP0 | EDMA_REQ_PORTA | EDMA_REQ_PORTB | EDMA_REQ_PORTC | EDMA_REQ_PORTD | EDMA_REQ_PORTE | EDMA_REQ_FLEXCAN0 | EDMA_REQ_FLEXCAN1 | EDMA_REQ_LPTMR0 | EDMA_REQ_DMAMUX_ALWAYS_ENABLED0 | EDMA_REQ_DMAMUX_ALWAYS_ENABLED1
      mask Callback channel11enable: mbd_s32k_edma_config_en_chn()
      mask TypeOptions channel12priority: EDMA_CHN_DEFAULT_PRIORITY | EDMA_CHN_PRIORITY_0 | EDMA_CHN_PRIORITY_1 | EDMA_CHN_PRIORITY_2 | EDMA_CHN_PRIORITY_3 | EDMA_CHN_PRIORITY_4 | EDMA_CHN_PRIORITY_5 | EDMA_CHN_PRIORITY_6 | EDMA_CHN_PRIORITY_7 | EDMA_CHN_PRIORITY_8 | EDMA_CHN_PRIORITY_9 | EDMA_CHN_PRIORITY_10 | EDMA_CHN_PRIORITY_11 | EDMA_CHN_PRIORITY_12 | EDMA_CHN_PRIORITY_13 | EDMA_CHN_PRIORITY_14 | EDMA_CHN_PRIORITY_15
      mask Callback channel12priority: mbd_s32k_edma_transfer_priority_cbk('12')
      mask TypeOptions channel12requestsource: EDMA_REQ_DISABLED | EDMA_REQ_LPUART0_RX | EDMA_REQ_LPUART0_TX | EDMA_REQ_LPUART1_RX | EDMA_REQ_LPUART1_TX | EDMA_REQ_FLEXIO_SHIFTER0 | EDMA_REQ_FLEXIO_SHIFTER1 | EDMA_REQ_FLEXIO_SHIFTER2 | EDMA_REQ_FLEXIO_SHIFTER3 | EDMA_REQ_LPSPI0_RX | EDMA_REQ_LPSPI0_TX | EDMA_REQ_LPSPI1_RX | EDMA_REQ_LPSPI1_TX | EDMA_REQ_FTM1_CHANNEL_0 | EDMA_REQ_FTM1_CHANNEL_1 | EDMA_REQ_FTM1_CHANNEL_2 | EDMA_REQ_FTM1_CHANNEL_3 | EDMA_REQ_FTM1_CHANNEL_4 | EDMA_REQ_FTM1_CHANNEL_5 | EDMA_REQ_FTM1_CHANNEL_6 | EDMA_REQ_FTM1_CHANNEL_7 | EDMA_REQ_FTM2_CHANNEL_0 | EDMA_REQ_FTM2_CHANNEL_1 | EDMA_REQ_FTM2_CHANNEL_2 | EDMA_REQ_FTM2_CHANNEL_3 | EDMA_REQ_FTM2_CHANNEL_4 | EDMA_REQ_FTM2_CHANNEL_5 | EDMA_REQ_FTM2_CHANNEL_6 | EDMA_REQ_FTM2_CHANNEL_7 | EDMA_REQ_FTM0_OR_CH0_CH7 | EDMA_REQ_FTM3_OR_CH0_CH7 | EDMA_REQ_ADC0 | EDMA_REQ_ADC1 | EDMA_REQ_LPI2C0_RX | EDMA_REQ_LPI2C0_TX | EDMA_REQ_PDB0 | EDMA_REQ_PDB1 | EDMA_REQ_CMP0 | EDMA_REQ_PORTA | EDMA_REQ_PORTB | EDMA_REQ_PORTC | EDMA_REQ_PORTD | EDMA_REQ_PORTE | EDMA_REQ_FLEXCAN0 | EDMA_REQ_FLEXCAN1 | EDMA_REQ_LPTMR0 | EDMA_REQ_DMAMUX_ALWAYS_ENABLED0 | EDMA_REQ_DMAMUX_ALWAYS_ENABLED1
      mask Callback channel12enable: mbd_s32k_edma_config_en_chn()
      mask TypeOptions channel13priority: EDMA_CHN_DEFAULT_PRIORITY | EDMA_CHN_PRIORITY_0 | EDMA_CHN_PRIORITY_1 | EDMA_CHN_PRIORITY_2 | EDMA_CHN_PRIORITY_3 | EDMA_CHN_PRIORITY_4 | EDMA_CHN_PRIORITY_5 | EDMA_CHN_PRIORITY_6 | EDMA_CHN_PRIORITY_7 | EDMA_CHN_PRIORITY_8 | EDMA_CHN_PRIORITY_9 | EDMA_CHN_PRIORITY_10 | EDMA_CHN_PRIORITY_11 | EDMA_CHN_PRIORITY_12 | EDMA_CHN_PRIORITY_13 | EDMA_CHN_PRIORITY_14 | EDMA_CHN_PRIORITY_15
      mask Callback channel13priority: mbd_s32k_edma_transfer_priority_cbk('13')
      mask TypeOptions channel13requestsource: EDMA_REQ_DISABLED | EDMA_REQ_LPUART0_RX | EDMA_REQ_LPUART0_TX | EDMA_REQ_LPUART1_RX | EDMA_REQ_LPUART1_TX | EDMA_REQ_FLEXIO_SHIFTER0 | EDMA_REQ_FLEXIO_SHIFTER1 | EDMA_REQ_FLEXIO_SHIFTER2 | EDMA_REQ_FLEXIO_SHIFTER3 | EDMA_REQ_LPSPI0_RX | EDMA_REQ_LPSPI0_TX | EDMA_REQ_LPSPI1_RX | EDMA_REQ_LPSPI1_TX | EDMA_REQ_FTM1_CHANNEL_0 | EDMA_REQ_FTM1_CHANNEL_1 | EDMA_REQ_FTM1_CHANNEL_2 | EDMA_REQ_FTM1_CHANNEL_3 | EDMA_REQ_FTM1_CHANNEL_4 | EDMA_REQ_FTM1_CHANNEL_5 | EDMA_REQ_FTM1_CHANNEL_6 | EDMA_REQ_FTM1_CHANNEL_7 | EDMA_REQ_FTM2_CHANNEL_0 | EDMA_REQ_FTM2_CHANNEL_1 | EDMA_REQ_FTM2_CHANNEL_2 | EDMA_REQ_FTM2_CHANNEL_3 | EDMA_REQ_FTM2_CHANNEL_4 | EDMA_REQ_FTM2_CHANNEL_5 | EDMA_REQ_FTM2_CHANNEL_6 | EDMA_REQ_FTM2_CHANNEL_7 | EDMA_REQ_FTM0_OR_CH0_CH7 | EDMA_REQ_FTM3_OR_CH0_CH7 | EDMA_REQ_ADC0 | EDMA_REQ_ADC1 | EDMA_REQ_LPI2C0_RX | EDMA_REQ_LPI2C0_TX | EDMA_REQ_PDB0 | EDMA_REQ_PDB1 | EDMA_REQ_CMP0 | EDMA_REQ_PORTA | EDMA_REQ_PORTB | EDMA_REQ_PORTC | EDMA_REQ_PORTD | EDMA_REQ_PORTE | EDMA_REQ_FLEXCAN0 | EDMA_REQ_FLEXCAN1 | EDMA_REQ_LPTMR0 | EDMA_REQ_DMAMUX_ALWAYS_ENABLED0 | EDMA_REQ_DMAMUX_ALWAYS_ENABLED1
      mask Callback channel13enable: mbd_s32k_edma_config_en_chn()
      mask TypeOptions channel14priority: EDMA_CHN_DEFAULT_PRIORITY | EDMA_CHN_PRIORITY_0 | EDMA_CHN_PRIORITY_1 | EDMA_CHN_PRIORITY_2 | EDMA_CHN_PRIORITY_3 | EDMA_CHN_PRIORITY_4 | EDMA_CHN_PRIORITY_5 | EDMA_CHN_PRIORITY_6 | EDMA_CHN_PRIORITY_7 | EDMA_CHN_PRIORITY_8 | EDMA_CHN_PRIORITY_9 | EDMA_CHN_PRIORITY_10 | EDMA_CHN_PRIORITY_11 | EDMA_CHN_PRIORITY_12 | EDMA_CHN_PRIORITY_13 | EDMA_CHN_PRIORITY_14 | EDMA_CHN_PRIORITY_15
      mask Callback channel14priority: mbd_s32k_edma_transfer_priority_cbk('14')
      mask TypeOptions channel14requestsource: EDMA_REQ_DISABLED | EDMA_REQ_LPUART0_RX | EDMA_REQ_LPUART0_TX | EDMA_REQ_LPUART1_RX | EDMA_REQ_LPUART1_TX | EDMA_REQ_FLEXIO_SHIFTER0 | EDMA_REQ_FLEXIO_SHIFTER1 | EDMA_REQ_FLEXIO_SHIFTER2 | EDMA_REQ_FLEXIO_SHIFTER3 | EDMA_REQ_LPSPI0_RX | EDMA_REQ_LPSPI0_TX | EDMA_REQ_LPSPI1_RX | EDMA_REQ_LPSPI1_TX | EDMA_REQ_FTM1_CHANNEL_0 | EDMA_REQ_FTM1_CHANNEL_1 | EDMA_REQ_FTM1_CHANNEL_2 | EDMA_REQ_FTM1_CHANNEL_3 | EDMA_REQ_FTM1_CHANNEL_4 | EDMA_REQ_FTM1_CHANNEL_5 | EDMA_REQ_FTM1_CHANNEL_6 | EDMA_REQ_FTM1_CHANNEL_7 | EDMA_REQ_FTM2_CHANNEL_0 | EDMA_REQ_FTM2_CHANNEL_1 | EDMA_REQ_FTM2_CHANNEL_2 | EDMA_REQ_FTM2_CHANNEL_3 | EDMA_REQ_FTM2_CHANNEL_4 | EDMA_REQ_FTM2_CHANNEL_5 | EDMA_REQ_FTM2_CHANNEL_6 | EDMA_REQ_FTM2_CHANNEL_7 | EDMA_REQ_FTM0_OR_CH0_CH7 | EDMA_REQ_FTM3_OR_CH0_CH7 | EDMA_REQ_ADC0 | EDMA_REQ_ADC1 | EDMA_REQ_LPI2C0_RX | EDMA_REQ_LPI2C0_TX | EDMA_REQ_PDB0 | EDMA_REQ_PDB1 | EDMA_REQ_CMP0 | EDMA_REQ_PORTA | EDMA_REQ_PORTB | EDMA_REQ_PORTC | EDMA_REQ_PORTD | EDMA_REQ_PORTE | EDMA_REQ_FLEXCAN0 | EDMA_REQ_FLEXCAN1 | EDMA_REQ_LPTMR0 | EDMA_REQ_DMAMUX_ALWAYS_ENABLED0 | EDMA_REQ_DMAMUX_ALWAYS_ENABLED1
      mask Callback channel14enable: mbd_s32k_edma_config_en_chn()
      mask TypeOptions channel15priority: EDMA_CHN_DEFAULT_PRIORITY | EDMA_CHN_PRIORITY_0 | EDMA_CHN_PRIORITY_1 | EDMA_CHN_PRIORITY_2 | EDMA_CHN_PRIORITY_3 | EDMA_CHN_PRIORITY_4 | EDMA_CHN_PRIORITY_5 | EDMA_CHN_PRIORITY_6 | EDMA_CHN_PRIORITY_7 | EDMA_CHN_PRIORITY_8 | EDMA_CHN_PRIORITY_9 | EDMA_CHN_PRIORITY_10 | EDMA_CHN_PRIORITY_11 | EDMA_CHN_PRIORITY_12 | EDMA_CHN_PRIORITY_13 | EDMA_CHN_PRIORITY_14 | EDMA_CHN_PRIORITY_15
      mask Callback channel15priority: mbd_s32k_edma_transfer_priority_cbk('15')
      mask TypeOptions channel15requestsource: EDMA_REQ_DISABLED | EDMA_REQ_LPUART0_RX | EDMA_REQ_LPUART0_TX | EDMA_REQ_LPUART1_RX | EDMA_REQ_LPUART1_TX | EDMA_REQ_FLEXIO_SHIFTER0 | EDMA_REQ_FLEXIO_SHIFTER1 | EDMA_REQ_FLEXIO_SHIFTER2 | EDMA_REQ_FLEXIO_SHIFTER3 | EDMA_REQ_LPSPI0_RX | EDMA_REQ_LPSPI0_TX | EDMA_REQ_LPSPI1_RX | EDMA_REQ_LPSPI1_TX | EDMA_REQ_FTM1_CHANNEL_0 | EDMA_REQ_FTM1_CHANNEL_1 | EDMA_REQ_FTM1_CHANNEL_2 | EDMA_REQ_FTM1_CHANNEL_3 | EDMA_REQ_FTM1_CHANNEL_4 | EDMA_REQ_FTM1_CHANNEL_5 | EDMA_REQ_FTM1_CHANNEL_6 | EDMA_REQ_FTM1_CHANNEL_7 | EDMA_REQ_FTM2_CHANNEL_0 | EDMA_REQ_FTM2_CHANNEL_1 | EDMA_REQ_FTM2_CHANNEL_2 | EDMA_REQ_FTM2_CHANNEL_3 | EDMA_REQ_FTM2_CHANNEL_4 | EDMA_REQ_FTM2_CHANNEL_5 | EDMA_REQ_FTM2_CHANNEL_6 | EDMA_REQ_FTM2_CHANNEL_7 | EDMA_REQ_FTM0_OR_CH0_CH7 | EDMA_REQ_FTM3_OR_CH0_CH7 | EDMA_REQ_ADC0 | EDMA_REQ_ADC1 | EDMA_REQ_LPI2C0_RX | EDMA_REQ_LPI2C0_TX | EDMA_REQ_PDB0 | EDMA_REQ_PDB1 | EDMA_REQ_CMP0 | EDMA_REQ_PORTA | EDMA_REQ_PORTB | EDMA_REQ_PORTC | EDMA_REQ_PORTD | EDMA_REQ_PORTE | EDMA_REQ_FLEXCAN0 | EDMA_REQ_FLEXCAN1 | EDMA_REQ_LPTMR0 | EDMA_REQ_DMAMUX_ALWAYS_ENABLED0 | EDMA_REQ_DMAMUX_ALWAYS_ENABLED1
      mask Callback channel15enable: mbd_s32k_edma_config_en_chn()
      mask Display:
      | image('nxp_logo.png', 'top-right');
      | disp(maskStr);
  eDMA_Transfer : S-Function  FunctionName=edma_s32k_transfer  Parameters=sFuncParams  SFunctionDeploymentMode=off  EnableBusSupport=off  mask(edma_s32k_transfer){channel=0, transfer_mode=Scatter-Gather Transfer, transfer_type=EDMA_TRANSFER_MEM2MEM, transfer_size=EDMA_TRANSFER_SIZE_1B, single_block_src_type=Src input is an address, single_block_dest_type=Dest input is an address, bytes_on_each_req=8, sg_struct_size=8, src_list={0x0,0x0}, src_list_type=Address list, dest_list={0x0,0x0}, dest_list_type=Address list, src_periph1=ADC0, src_reg1=SC1A, src_reg1offset=0, src_reg1enable=off, src_reg1_addr=0x4003B000, src_periph2=ADC0, src_reg2=SC1A, src_reg2offset=0, src_reg2enable=off, src_reg2_addr=0x4003B000, src_periph3=ADC0, src_reg3=SC1A, src_reg3offset=0, src_reg3enable=off, src_reg3_addr=0x4003B000, src_periph4=ADC0, src_reg4=SC1A, src_reg4offset=0, src_reg4enable=off, src_reg4_addr=0x4003B000, src_periph5=ADC0, src_reg5=SC1A, src_reg5offset=0, src_reg5enable=off, src_reg5_addr=0x4003B000, src_periph6=ADC0, src_reg6=SC1A, src_reg6offset=0, src_reg6enable=off, src_reg6_addr=0x4003B000, src_periph7=ADC0, src_reg7=SC1A, src_reg7offset=0, src_reg7enable=off, src_reg7_addr=0x4003B000, src_periph8=ADC0, src_reg8=SC1A, src_reg8offset=0, src_reg8enable=off, src_reg8_addr=0x4003B000, dest_periph1=ADC0, dest_reg1=SC1A, dest_reg1offset=0, dest_reg1enable=off, dest_reg1_addr=0x4003B000, dest_periph2=ADC0, dest_reg2=SC1A, dest_reg2offset=0, dest_reg2enable=off, dest_reg2_addr=0x4003B000, dest_periph3=ADC0, dest_reg3=SC1A, dest_reg3offset=0, dest_reg3enable=off, dest_reg3_addr=0x4003B000, dest_periph4=ADC0, dest_reg4=SC1A, dest_reg4offset=0, dest_reg4enable=off, dest_reg4_addr=0x4003B000, dest_periph5=ADC0, dest_reg5=SC1A, dest_reg5offset=0, dest_reg5enable=off, dest_reg5_addr=0x4003B000, dest_periph6=ADC0, dest_reg6=SC1A, dest_reg6offset=0, dest_reg6enable=off, dest_reg6_addr=0x4003B000, dest_periph7=ADC0, dest_reg7=SC1A, dest_reg7offset=0, dest_reg7enable=off, dest_reg7_addr=0x4003B000, dest_periph8=ADC0, dest_reg8=SC1A, dest_reg8offset=0, dest_reg8enable=off, dest_reg8_addr=0x4003B000}
      mask prompts: transfer_mode "Transfer mode"; transfer_type "Transfer type"; transfer_size "Transfer size"; single_block_src_type "Src input type"; single_block_dest_type "Dest input type"; bytes_on_each_req "Bytes on each request"; sg_struct_size "Src/Dest width (bits)"; src_list "Source List"; dest_list "Destination List"; src_periph1 "Peripheral"; src_reg1 "Register"; src_reg1offset "Offset"; src_reg1enable "Use"; src_reg1_addr "addr"; src_periph2 "Peripheral"; src_reg2 "Register"; src_reg2offset "Offset"; src_reg2enable "Use"; src_reg2_addr "addr"; src_periph3 "Peripheral"; src_reg3 "Register"; src_reg3offset "Offset"; src_reg3enable "Use"; src_reg3_addr "addr"; src_periph4 "Peripheral"; src_reg4 "Register"; src_reg4offset "Offset"; src_reg4enable "Use"; src_reg4_addr "addr"; src_periph5 "Peripheral"; src_reg5 "Register"; src_reg5offset "Offset"; src_reg5enable "Use"; src_reg5_addr "addr"; src_periph6 "Peripheral"; src_reg6 "Register"; src_reg6offset "Offset"; src_reg6enable "Use"; src_reg6_addr "addr"; src_periph7 "Peripheral"; src_reg7 "Register"; src_reg7offset "Offset"; src_reg7enable "Use"; src_reg7_addr "addr"; src_periph8 "Peripheral"; src_reg8 "Register"; src_reg8offset "Offset"; src_reg8enable "Use"; src_reg8_addr "addr"; dest_periph1 "Peripheral"; dest_reg1 "Register"; dest_reg1offset "Offset"; dest_reg1enable "Use"; dest_reg1_addr "addr"; dest_periph2 "Peripheral"; dest_reg2 "Register"; dest_reg2offset "Offset"; dest_reg2enable "Use"; dest_reg2_addr "addr"; dest_periph3 "Peripheral"; dest_reg3 "Register"; dest_reg3offset "Offset"; dest_reg3enable "Use"; dest_reg3_addr "addr"; dest_periph4 "Peripheral"; dest_reg4 "Register"; dest_reg4offset "Offset"; dest_reg4enable "Use"; dest_reg4_addr "addr"; dest_periph5 "Peripheral"; dest_reg5 "Register"; dest_reg5offset "Offset"; dest_reg5enable "Use"; dest_reg5_addr "addr"; dest_periph6 "Peripheral"; dest_reg6 "Register"; dest_reg6offset "Offset"; dest_reg6enable "Use"; dest_reg6_addr "addr"; dest_periph7 "Peripheral"; dest_reg7 "Register"; dest_reg7offset "Offset"; dest_reg7enable "Use"; dest_reg7_addr "addr"; dest_periph8 "Peripheral"; dest_reg8 "Register"; dest_reg8offset "Offset"; dest_reg8enable "Use"; dest_reg8_addr "addr"
      mask help: This block allows the user to transfer data via eDMA.
      mask init:
      | [maskStr, sFuncParams] = mbd_s32k_edma_transfer();
      settings: NameChangeFcn=mbd_s32k_name_check(gcb);
      mask Help: web(fullfile(mbd_s32k_block_help, 'edma', 'edma_transfer.html'));
      mask TypeOptions channel: 0 | 1 | 2 | 3 | 4 | 5 | 6 | 7 | 8 | 9 | 10 | 11 | 12 | 13 | 14 | 15
      mask TypeOptions transfer_mode: Single Block Transfer | Scatter-Gather Transfer
      mask Callback transfer_mode: mbd_s32k_edma_transfer_mode_cbk()
      mask TypeOptions transfer_type: EDMA_TRANSFER_MEM2MEM | EDMA_TRANSFER_PERIPH2MEM | EDMA_TRANSFER_MEM2PERIPH | EDMA_TRANSFER_PERIPH2PERIPH
      mask TypeOptions transfer_size: EDMA_TRANSFER_SIZE_1B | EDMA_TRANSFER_SIZE_2B | EDMA_TRANSFER_SIZE_4B | EDMA_TRANSFER_SIZE_16B | EDMA_TRANSFER_SIZE_32B
      mask Callback transfer_size: mbd_s32k_edma_transfer_size_cbk()
      mask TypeOptions single_block_src_type: Src input is an address | Src input is a variable (data)
      mask TypeOptions single_block_dest_type: Dest input is an address | Dest input is a variable (data)
      mask Callback bytes_on_each_req: mbd_s32k_edma_transfer_mode_cbk()
      mask Callback sg_struct_size: mbd_s32k_edma_transfer_mode_cbk()
      mask Callback src_list: mbd_s32k_edma_transfer_mode_cbk()
      mask TypeOptions src_list_type: Address list | Value list | Select from a register list
      mask Callback src_list_type: mbd_s32k_edma_list_type_cbk('src')
      mask Callback dest_list: mbd_s32k_edma_transfer_mode_cbk()
      mask TypeOptions dest_list_type: Address list | Value list | Select from a register list
      mask Callback dest_list_type: mbd_s32k_edma_list_type_cbk('dest')
      mask TypeOptions src_periph1: ADC0 | ADC1 | AIPS | CAN0 | CAN1 | CAN2 | CMP0 | CRC | CSE_PRAM | DMA | DMAMUX | EIM | ENET | ERM | EWM | FLEXIO | FTFC | FTM0 | FTM1 | FTM2 | FTM3 | FTM4 | FTM5 | FTM6 | FTM7 | LMEM | LPI2C0 | LPI2C1 | LPIT0 | LPSPI0 | LPSPI1 | LPSPI2 | LPTMR0 | LPUART0 | LPUART1 | LPUART2 | MCM | MPU | MSCM | PCC | PDB0 | PDB1 | PMC | PORTA | PORTB | PORTC | PORTD | PORTE | PTA | PTB | PTC | PTD | PTE | Qu | RCM | RTC | S32_NVIC | S32_SCB | S32_SysTick | SAI0 | SAI1 | SCG | SIM | SMC | TRGMUX | WDOG
      mask Callback src_periph1: mbd_s32k_edma_periph_update_cbk('read','src','1')
      mask TypeOptions src_reg1: SC1A | SC1B | SC1C | SC1D | SC1E | SC1F | SC1G | SC1H | SC1I | SC1J | SC1K | SC1L | SC1M | SC1N | SC1O | SC1P | CFG1 | CFG2 | RA | RB | RC | RD | RE | RF | RG | RH | RI | RJ | RK | RL | RM | RN | RO | RP | CV1 | CV2 | SC2 | SC3 | BASE_OFS | OFS | USR_OFS | XOFS | YOFS | G | UG | CLPS | CLP3 | CLP2 | CLP1 | CLP0 | CLPX | CLP9 | CLPS_OFS | CLP3_OFS | CLP2_OFS | CLP1_OFS | CLP0_OFS | CLPX_OFS | CLP9_OFS | aSC1A | aSC1B | aSC1C | aSC1D | aSC1E | aSC1F | aSC1G | aSC1H | aSC1I | aSC1J | aSC1K | aSC1L | aSC1M | aSC1N | aSC1O | aSC1P | SC1Q | SC1R | SC1S | SC1T | SC1U | SC1V | SC1W | SC1X | SC1Y | SC1Z | SC1AA | SC1AB | SC1AC | SC1AD | SC1AE | SC1AF | aRA | aRB | aRC | aRD | aRE | aRF | aRG | aRH | aRI | aRJ | aRK | aRL | aRM | aRN | aRO | aRP | RQ | RR | RS | RT | RU | RV | RW | RX | RY | RZ | RAA | RAB | RAC | RAD | RAE | RAF
      mask Callback src_reg1: mbd_s32k_edma_reg_update_cbk('src','1')
      mask Callback src_reg1enable: mbd_s32k_edma_new_src_reg_cbk(1)
      mask TypeOptions src_periph2: ADC0 | ADC1 | AIPS | CAN0 | CAN1 | CAN2 | CMP0 | CRC | CSE_PRAM | DMA | DMAMUX | EIM | ENET | ERM | EWM | FLEXIO | FTFC | FTM0 | FTM1 | FTM2 | FTM3 | FTM4 | FTM5 | FTM6 | FTM7 | LMEM | LPI2C0 | LPI2C1 | LPIT0 | LPSPI0 | LPSPI1 | LPSPI2 | LPTMR0 | LPUART0 | LPUART1 | LPUART2 | MCM | MPU | MSCM | PCC | PDB0 | PDB1 | PMC | PORTA | PORTB | PORTC | PORTD | PORTE | PTA | PTB | PTC | PTD | PTE | Qu | RCM | RTC | S32_NVIC | S32_SCB | S32_SysTick | SAI0 | SAI1 | SCG | SIM | SMC | TRGMUX | WDOG
      mask Callback src_periph2: mbd_s32k_edma_periph_update_cbk('read','src','2')
      mask TypeOptions src_reg2: SC1A | SC1B | SC1C | SC1D | SC1E | SC1F | SC1G | SC1H | SC1I | SC1J | SC1K | SC1L | SC1M | SC1N | SC1O | SC1P | CFG1 | CFG2 | RA | RB | RC | RD | RE | RF | RG | RH | RI | RJ | RK | RL | RM | RN | RO | RP | CV1 | CV2 | SC2 | SC3 | BASE_OFS | OFS | USR_OFS | XOFS | YOFS | G | UG | CLPS | CLP3 | CLP2 | CLP1 | CLP0 | CLPX | CLP9 | CLPS_OFS | CLP3_OFS | CLP2_OFS | CLP1_OFS | CLP0_OFS | CLPX_OFS | CLP9_OFS | aSC1A | aSC1B | aSC1C | aSC1D | aSC1E | aSC1F | aSC1G | aSC1H | aSC1I | aSC1J | aSC1K | aSC1L | aSC1M | aSC1N | aSC1O | aSC1P | SC1Q | SC1R | SC1S | SC1T | SC1U | SC1V | SC1W | SC1X | SC1Y | SC1Z | SC1AA | SC1AB | SC1AC | SC1AD | SC1AE | SC1AF | aRA | aRB | aRC | aRD | aRE | aRF | aRG | aRH | aRI | aRJ | aRK | aRL | aRM | aRN | aRO | aRP | RQ | RR | RS | RT | RU | RV | RW | RX | RY | RZ | RAA | RAB | RAC | RAD | RAE | RAF
      mask Callback src_reg2: mbd_s32k_edma_reg_update_cbk('src','2')
      mask Callback src_reg2enable: mbd_s32k_edma_new_src_reg_cbk(2)
      mask TypeOptions src_periph3: ADC0 | ADC1 | AIPS | CAN0 | CAN1 | CAN2 | CMP0 | CRC | CSE_PRAM | DMA | DMAMUX | EIM | ENET | ERM | EWM | FLEXIO | FTFC | FTM0 | FTM1 | FTM2 | FTM3 | FTM4 | FTM5 | FTM6 | FTM7 | LMEM | LPI2C0 | LPI2C1 | LPIT0 | LPSPI0 | LPSPI1 | LPSPI2 | LPTMR0 | LPUART0 | LPUART1 | LPUART2 | MCM | MPU | MSCM | PCC | PDB0 | PDB1 | PMC | PORTA | PORTB | PORTC | PORTD | PORTE | PTA | PTB | PTC | PTD | PTE | Qu | RCM | RTC | S32_NVIC | S32_SCB | S32_SysTick | SAI0 | SAI1 | SCG | SIM | SMC | TRGMUX | WDOG
      mask Callback src_periph3: mbd_s32k_edma_periph_update_cbk('read','src','3')
      mask TypeOptions src_reg3: SC1A | SC1B | SC1C | SC1D | SC1E | SC1F | SC1G | SC1H | SC1I | SC1J | SC1K | SC1L | SC1M | SC1N | SC1O | SC1P | CFG1 | CFG2 | RA | RB | RC | RD | RE | RF | RG | RH | RI | RJ | RK | RL | RM | RN | RO | RP | CV1 | CV2 | SC2 | SC3 | BASE_OFS | OFS | USR_OFS | XOFS | YOFS | G | UG | CLPS | CLP3 | CLP2 | CLP1 | CLP0 | CLPX | CLP9 | CLPS_OFS | CLP3_OFS | CLP2_OFS | CLP1_OFS | CLP0_OFS | CLPX_OFS | CLP9_OFS | aSC1A | aSC1B | aSC1C | aSC1D | aSC1E | aSC1F | aSC1G | aSC1H | aSC1I | aSC1J | aSC1K | aSC1L | aSC1M | aSC1N | aSC1O | aSC1P | SC1Q | SC1R | SC1S | SC1T | SC1U | SC1V | SC1W | SC1X | SC1Y | SC1Z | SC1AA | SC1AB | SC1AC | SC1AD | SC1AE | SC1AF | aRA | aRB | aRC | aRD | aRE | aRF | aRG | aRH | aRI | aRJ | aRK | aRL | aRM | aRN | aRO | aRP | RQ | RR | RS | RT | RU | RV | RW | RX | RY | RZ | RAA | RAB | RAC | RAD | RAE | RAF
      mask Callback src_reg3: mbd_s32k_edma_reg_update_cbk('src','3')
      mask Callback src_reg3enable: mbd_s32k_edma_new_src_reg_cbk(3)
      mask TypeOptions src_periph4: ADC0 | ADC1 | AIPS | CAN0 | CAN1 | CAN2 | CMP0 | CRC | CSE_PRAM | DMA | DMAMUX | EIM | ENET | ERM | EWM | FLEXIO | FTFC | FTM0 | FTM1 | FTM2 | FTM3 | FTM4 | FTM5 | FTM6 | FTM7 | LMEM | LPI2C0 | LPI2C1 | LPIT0 | LPSPI0 | LPSPI1 | LPSPI2 | LPTMR0 | LPUART0 | LPUART1 | LPUART2 | MCM | MPU | MSCM | PCC | PDB0 | PDB1 | PMC | PORTA | PORTB | PORTC | PORTD | PORTE | PTA | PTB | PTC | PTD | PTE | Qu | RCM | RTC | S32_NVIC | S32_SCB | S32_SysTick | SAI0 | SAI1 | SCG | SIM | SMC | TRGMUX | WDOG
      mask Callback src_periph4: mbd_s32k_edma_periph_update_cbk('read','src','4')
      mask TypeOptions src_reg4: SC1A | SC1B | SC1C | SC1D | SC1E | SC1F | SC1G | SC1H | SC1I | SC1J | SC1K | SC1L | SC1M | SC1N | SC1O | SC1P | CFG1 | CFG2 | RA | RB | RC | RD | RE | RF | RG | RH | RI | RJ | RK | RL | RM | RN | RO | RP | CV1 | CV2 | SC2 | SC3 | BASE_OFS | OFS | USR_OFS | XOFS | YOFS | G | UG | CLPS | CLP3 | CLP2 | CLP1 | CLP0 | CLPX | CLP9 | CLPS_OFS | CLP3_OFS | CLP2_OFS | CLP1_OFS | CLP0_OFS | CLPX_OFS | CLP9_OFS | aSC1A | aSC1B | aSC1C | aSC1D | aSC1E | aSC1F | aSC1G | aSC1H | aSC1I | aSC1J | aSC1K | aSC1L | aSC1M | aSC1N | aSC1O | aSC1P | SC1Q | SC1R | SC1S | SC1T | SC1U | SC1V | SC1W | SC1X | SC1Y | SC1Z | SC1AA | SC1AB | SC1AC | SC1AD | SC1AE | SC1AF | aRA | aRB | aRC | aRD | aRE | aRF | aRG | aRH | aRI | aRJ | aRK | aRL | aRM | aRN | aRO | aRP | RQ | RR | RS | RT | RU | RV | RW | RX | RY | RZ | RAA | RAB | RAC | RAD | RAE | RAF
      mask Callback src_reg4: mbd_s32k_edma_reg_update_cbk('src','4')
      mask Callback src_reg4enable: mbd_s32k_edma_new_src_reg_cbk(4)
      mask TypeOptions src_periph5: ADC0 | ADC1 | AIPS | CAN0 | CAN1 | CAN2 | CMP0 | CRC | CSE_PRAM | DMA | DMAMUX | EIM | ENET | ERM | EWM | FLEXIO | FTFC | FTM0 | FTM1 | FTM2 | FTM3 | FTM4 | FTM5 | FTM6 | FTM7 | LMEM | LPI2C0 | LPI2C1 | LPIT0 | LPSPI0 | LPSPI1 | LPSPI2 | LPTMR0 | LPUART0 | LPUART1 | LPUART2 | MCM | MPU | MSCM | PCC | PDB0 | PDB1 | PMC | PORTA | PORTB | PORTC | PORTD | PORTE | PTA | PTB | PTC | PTD | PTE | Qu | RCM | RTC | S32_NVIC | S32_SCB | S32_SysTick | SAI0 | SAI1 | SCG | SIM | SMC | TRGMUX | WDOG
      mask Callback src_periph5: mbd_s32k_edma_periph_update_cbk('read','src','5')
      mask TypeOptions src_reg5: SC1A | SC1B | SC1C | SC1D | SC1E | SC1F | SC1G | SC1H | SC1I | SC1J | SC1K | SC1L | SC1M | SC1N | SC1O | SC1P | CFG1 | CFG2 | RA | RB | RC | RD | RE | RF | RG | RH | RI | RJ | RK | RL | RM | RN | RO | RP | CV1 | CV2 | SC2 | SC3 | BASE_OFS | OFS | USR_OFS | XOFS | YOFS | G | UG | CLPS | CLP3 | CLP2 | CLP1 | CLP0 | CLPX | CLP9 | CLPS_OFS | CLP3_OFS | CLP2_OFS | CLP1_OFS | CLP0_OFS | CLPX_OFS | CLP9_OFS | aSC1A | aSC1B | aSC1C | aSC1D | aSC1E | aSC1F | aSC1G | aSC1H | aSC1I | aSC1J | aSC1K | aSC1L | aSC1M | aSC1N | aSC1O | aSC1P | SC1Q | SC1R | SC1S | SC1T | SC1U | SC1V | SC1W | SC1X | SC1Y | SC1Z | SC1AA | SC1AB | SC1AC | SC1AD | SC1AE | SC1AF | aRA | aRB | aRC | aRD | aRE | aRF | aRG | aRH | aRI | aRJ | aRK | aRL | aRM | aRN | aRO | aRP | RQ | RR | RS | RT | RU | RV | RW | RX | RY | RZ | RAA | RAB | RAC | RAD | RAE | RAF
      mask Callback src_reg5: mbd_s32k_edma_reg_update_cbk('src','5')
      mask Callback src_reg5enable: mbd_s32k_edma_new_src_reg_cbk(5)
      mask TypeOptions src_periph6: ADC0 | ADC1 | AIPS | CAN0 | CAN1 | CAN2 | CMP0 | CRC | CSE_PRAM | DMA | DMAMUX | EIM | ENET | ERM | EWM | FLEXIO | FTFC | FTM0 | FTM1 | FTM2 | FTM3 | FTM4 | FTM5 | FTM6 | FTM7 | LMEM | LPI2C0 | LPI2C1 | LPIT0 | LPSPI0 | LPSPI1 | LPSPI2 | LPTMR0 | LPUART0 | LPUART1 | LPUART2 | MCM | MPU | MSCM | PCC | PDB0 | PDB1 | PMC | PORTA | PORTB | PORTC | PORTD | PORTE | PTA | PTB | PTC | PTD | PTE | Qu | RCM | RTC | S32_NVIC | S32_SCB | S32_SysTick | SAI0 | SAI1 | SCG | SIM | SMC | TRGMUX | WDOG
      mask Callback src_periph6: mbd_s32k_edma_periph_update_cbk('read','src','6')
      mask TypeOptions src_reg6: SC1A | SC1B | SC1C | SC1D | SC1E | SC1F | SC1G | SC1H | SC1I | SC1J | SC1K | SC1L | SC1M | SC1N | SC1O | SC1P | CFG1 | CFG2 | RA | RB | RC | RD | RE | RF | RG | RH | RI | RJ | RK | RL | RM | RN | RO | RP | CV1 | CV2 | SC2 | SC3 | BASE_OFS | OFS | USR_OFS | XOFS | YOFS | G | UG | CLPS | CLP3 | CLP2 | CLP1 | CLP0 | CLPX | CLP9 | CLPS_OFS | CLP3_OFS | CLP2_OFS | CLP1_OFS | CLP0_OFS | CLPX_OFS | CLP9_OFS | aSC1A | aSC1B | aSC1C | aSC1D | aSC1E | aSC1F | aSC1G | aSC1H | aSC1I | aSC1J | aSC1K | aSC1L | aSC1M | aSC1N | aSC1O | aSC1P | SC1Q | SC1R | SC1S | SC1T | SC1U | SC1V | SC1W | SC1X | SC1Y | SC1Z | SC1AA | SC1AB | SC1AC | SC1AD | SC1AE | SC1AF | aRA | aRB | aRC | aRD | aRE | aRF | aRG | aRH | aRI | aRJ | aRK | aRL | aRM | aRN | aRO | aRP | RQ | RR | RS | RT | RU | RV | RW | RX | RY | RZ | RAA | RAB | RAC | RAD | RAE | RAF
      mask Callback src_reg6: mbd_s32k_edma_reg_update_cbk('src','6')
      mask Callback src_reg6enable: mbd_s32k_edma_new_src_reg_cbk(6)
      mask TypeOptions src_periph7: ADC0 | ADC1 | AIPS | CAN0 | CAN1 | CAN2 | CMP0 | CRC | CSE_PRAM | DMA | DMAMUX | EIM | ENET | ERM | EWM | FLEXIO | FTFC | FTM0 | FTM1 | FTM2 | FTM3 | FTM4 | FTM5 | FTM6 | FTM7 | LMEM | LPI2C0 | LPI2C1 | LPIT0 | LPSPI0 | LPSPI1 | LPSPI2 | LPTMR0 | LPUART0 | LPUART1 | LPUART2 | MCM | MPU | MSCM | PCC | PDB0 | PDB1 | PMC | PORTA | PORTB | PORTC | PORTD | PORTE | PTA | PTB | PTC | PTD | PTE | Qu | RCM | RTC | S32_NVIC | S32_SCB | S32_SysTick | SAI0 | SAI1 | SCG | SIM | SMC | TRGMUX | WDOG
      mask Callback src_periph7: mbd_s32k_edma_periph_update_cbk('read','src','7')
      mask TypeOptions src_reg7: SC1A | SC1B | SC1C | SC1D | SC1E | SC1F | SC1G | SC1H | SC1I | SC1J | SC1K | SC1L | SC1M | SC1N | SC1O | SC1P | CFG1 | CFG2 | RA | RB | RC | RD | RE | RF | RG | RH | RI | RJ | RK | RL | RM | RN | RO | RP | CV1 | CV2 | SC2 | SC3 | BASE_OFS | OFS | USR_OFS | XOFS | YOFS | G | UG | CLPS | CLP3 | CLP2 | CLP1 | CLP0 | CLPX | CLP9 | CLPS_OFS | CLP3_OFS | CLP2_OFS | CLP1_OFS | CLP0_OFS | CLPX_OFS | CLP9_OFS | aSC1A | aSC1B | aSC1C | aSC1D | aSC1E | aSC1F | aSC1G | aSC1H | aSC1I | aSC1J | aSC1K | aSC1L | aSC1M | aSC1N | aSC1O | aSC1P | SC1Q | SC1R | SC1S | SC1T | SC1U | SC1V | SC1W | SC1X | SC1Y | SC1Z | SC1AA | SC1AB | SC1AC | SC1AD | SC1AE | SC1AF | aRA | aRB | aRC | aRD | aRE | aRF | aRG | aRH | aRI | aRJ | aRK | aRL | aRM | aRN | aRO | aRP | RQ | RR | RS | RT | RU | RV | RW | RX | RY | RZ | RAA | RAB | RAC | RAD | RAE | RAF
      mask Callback src_reg7: mbd_s32k_edma_reg_update_cbk('src','7')
      mask Callback src_reg7enable: mbd_s32k_edma_new_src_reg_cbk(7)
      mask TypeOptions src_periph8: ADC0 | ADC1 | AIPS | CAN0 | CAN1 | CAN2 | CMP0 | CRC | CSE_PRAM | DMA | DMAMUX | EIM | ENET | ERM | EWM | FLEXIO | FTFC | FTM0 | FTM1 | FTM2 | FTM3 | FTM4 | FTM5 | FTM6 | FTM7 | LMEM | LPI2C0 | LPI2C1 | LPIT0 | LPSPI0 | LPSPI1 | LPSPI2 | LPTMR0 | LPUART0 | LPUART1 | LPUART2 | MCM | MPU | MSCM | PCC | PDB0 | PDB1 | PMC | PORTA | PORTB | PORTC | PORTD | PORTE | PTA | PTB | PTC | PTD | PTE | Qu | RCM | RTC | S32_NVIC | S32_SCB | S32_SysTick | SAI0 | SAI1 | SCG | SIM | SMC | TRGMUX | WDOG
      mask Callback src_periph8: mbd_s32k_edma_periph_update_cbk('read','src','8')
      mask TypeOptions src_reg8: SC1A | SC1B | SC1C | SC1D | SC1E | SC1F | SC1G | SC1H | SC1I | SC1J | SC1K | SC1L | SC1M | SC1N | SC1O | SC1P | CFG1 | CFG2 | RA | RB | RC | RD | RE | RF | RG | RH | RI | RJ | RK | RL | RM | RN | RO | RP | CV1 | CV2 | SC2 | SC3 | BASE_OFS | OFS | USR_OFS | XOFS | YOFS | G | UG | CLPS | CLP3 | CLP2 | CLP1 | CLP0 | CLPX | CLP9 | CLPS_OFS | CLP3_OFS | CLP2_OFS | CLP1_OFS | CLP0_OFS | CLPX_OFS | CLP9_OFS | aSC1A | aSC1B | aSC1C | aSC1D | aSC1E | aSC1F | aSC1G | aSC1H | aSC1I | aSC1J | aSC1K | aSC1L | aSC1M | aSC1N | aSC1O | aSC1P | SC1Q | SC1R | SC1S | SC1T | SC1U | SC1V | SC1W | SC1X | SC1Y | SC1Z | SC1AA | SC1AB | SC1AC | SC1AD | SC1AE | SC1AF | aRA | aRB | aRC | aRD | aRE | aRF | aRG | aRH | aRI | aRJ | aRK | aRL | aRM | aRN | aRO | aRP | RQ | RR | RS | RT | RU | RV | RW | RX | RY | RZ | RAA | RAB | RAC | RAD | RAE | RAF
      mask Callback src_reg8: mbd_s32k_edma_reg_update_cbk('src','8')
      mask Callback src_reg8enable: mbd_s32k_edma_new_src_reg_cbk(8)
      mask TypeOptions dest_periph1: ADC0 | ADC1 | AIPS | CAN0 | CAN1 | CAN2 | CMP0 | CRC | CSE_PRAM | DMA | DMAMUX | EIM | ENET | ERM | EWM | FLEXIO | FTFC | FTM0 | FTM1 | FTM2 | FTM3 | FTM4 | FTM5 | FTM6 | FTM7 | LMEM | LPI2C0 | LPI2C1 | LPIT0 | LPSPI0 | LPSPI1 | LPSPI2 | LPTMR0 | LPUART0 | LPUART1 | LPUART2 | MCM | MPU | MSCM | PCC | PDB0 | PDB1 | PMC | PORTA | PORTB | PORTC | PORTD | PORTE | PTA | PTB | PTC | PTD | PTE | Qu | RCM | RTC | S32_NVIC | S32_SCB | S32_SysTick | SAI0 | SAI1 | SCG | SIM | SMC | TRGMUX | WDOG
      mask Callback dest_periph1: mbd_s32k_edma_periph_update_cbk('read','dest','1')
      mask TypeOptions dest_reg1: SC1A | SC1B | SC1C | SC1D | SC1E | SC1F | SC1G | SC1H | SC1I | SC1J | SC1K | SC1L | SC1M | SC1N | SC1O | SC1P | CFG1 | CFG2 | RA | RB | RC | RD | RE | RF | RG | RH | RI | RJ | RK | RL | RM | RN | RO | RP | CV1 | CV2 | SC2 | SC3 | BASE_OFS | OFS | USR_OFS | XOFS | YOFS | G | UG | CLPS | CLP3 | CLP2 | CLP1 | CLP0 | CLPX | CLP9 | CLPS_OFS | CLP3_OFS | CLP2_OFS | CLP1_OFS | CLP0_OFS | CLPX_OFS | CLP9_OFS | aSC1A | aSC1B | aSC1C | aSC1D | aSC1E | aSC1F | aSC1G | aSC1H | aSC1I | aSC1J | aSC1K | aSC1L | aSC1M | aSC1N | aSC1O | aSC1P | SC1Q | SC1R | SC1S | SC1T | SC1U | SC1V | SC1W | SC1X | SC1Y | SC1Z | SC1AA | SC1AB | SC1AC | SC1AD | SC1AE | SC1AF | aRA | aRB | aRC | aRD | aRE | aRF | aRG | aRH | aRI | aRJ | aRK | aRL | aRM | aRN | aRO | aRP | RQ | RR | RS | RT | RU | RV | RW | RX | RY | RZ | RAA | RAB | RAC | RAD | RAE | RAF
      mask Callback dest_reg1: mbd_s32k_edma_reg_update_cbk('dest','1')
      mask Callback dest_reg1enable: mbd_s32k_edma_new_dest_reg_cbk(1)
      mask TypeOptions dest_periph2: ADC0 | ADC1 | AIPS | CAN0 | CAN1 | CAN2 | CMP0 | CRC | CSE_PRAM | DMA | DMAMUX | EIM | ENET | ERM | EWM | FLEXIO | FTFC | FTM0 | FTM1 | FTM2 | FTM3 | FTM4 | FTM5 | FTM6 | FTM7 | LMEM | LPI2C0 | LPI2C1 | LPIT0 | LPSPI0 | LPSPI1 | LPSPI2 | LPTMR0 | LPUART0 | LPUART1 | LPUART2 | MCM | MPU | MSCM | PCC | PDB0 | PDB1 | PMC | PORTA | PORTB | PORTC | PORTD | PORTE | PTA | PTB | PTC | PTD | PTE | Qu | RCM | RTC | S32_NVIC | S32_SCB | S32_SysTick | SAI0 | SAI1 | SCG | SIM | SMC | TRGMUX | WDOG
      mask Callback dest_periph2: mbd_s32k_edma_periph_update_cbk('read','dest','2')
      mask TypeOptions dest_reg2: SC1A | SC1B | SC1C | SC1D | SC1E | SC1F | SC1G | SC1H | SC1I | SC1J | SC1K | SC1L | SC1M | SC1N | SC1O | SC1P | CFG1 | CFG2 | RA | RB | RC | RD | RE | RF | RG | RH | RI | RJ | RK | RL | RM | RN | RO | RP | CV1 | CV2 | SC2 | SC3 | BASE_OFS | OFS | USR_OFS | XOFS | YOFS | G | UG | CLPS | CLP3 | CLP2 | CLP1 | CLP0 | CLPX | CLP9 | CLPS_OFS | CLP3_OFS | CLP2_OFS | CLP1_OFS | CLP0_OFS | CLPX_OFS | CLP9_OFS | aSC1A | aSC1B | aSC1C | aSC1D | aSC1E | aSC1F | aSC1G | aSC1H | aSC1I | aSC1J | aSC1K | aSC1L | aSC1M | aSC1N | aSC1O | aSC1P | SC1Q | SC1R | SC1S | SC1T | SC1U | SC1V | SC1W | SC1X | SC1Y | SC1Z | SC1AA | SC1AB | SC1AC | SC1AD | SC1AE | SC1AF | aRA | aRB | aRC | aRD | aRE | aRF | aRG | aRH | aRI | aRJ | aRK | aRL | aRM | aRN | aRO | aRP | RQ | RR | RS | RT | RU | RV | RW | RX | RY | RZ | RAA | RAB | RAC | RAD | RAE | RAF
      mask Callback dest_reg2: mbd_s32k_edma_reg_update_cbk('dest','2')
      mask Callback dest_reg2enable: mbd_s32k_edma_new_dest_reg_cbk(2)
      mask TypeOptions dest_periph3: ADC0 | ADC1 | AIPS | CAN0 | CAN1 | CAN2 | CMP0 | CRC | CSE_PRAM | DMA | DMAMUX | EIM | ENET | ERM | EWM | FLEXIO | FTFC | FTM0 | FTM1 | FTM2 | FTM3 | FTM4 | FTM5 | FTM6 | FTM7 | LMEM | LPI2C0 | LPI2C1 | LPIT0 | LPSPI0 | LPSPI1 | LPSPI2 | LPTMR0 | LPUART0 | LPUART1 | LPUART2 | MCM | MPU | MSCM | PCC | PDB0 | PDB1 | PMC | PORTA | PORTB | PORTC | PORTD | PORTE | PTA | PTB | PTC | PTD | PTE | Qu | RCM | RTC | S32_NVIC | S32_SCB | S32_SysTick | SAI0 | SAI1 | SCG | SIM | SMC | TRGMUX | WDOG
      mask Callback dest_periph3: mbd_s32k_edma_periph_update_cbk('read','dest','3')
      mask TypeOptions dest_reg3: SC1A | SC1B | SC1C | SC1D | SC1E | SC1F | SC1G | SC1H | SC1I | SC1J | SC1K | SC1L | SC1M | SC1N | SC1O | SC1P | CFG1 | CFG2 | RA | RB | RC | RD | RE | RF | RG | RH | RI | RJ | RK | RL | RM | RN | RO | RP | CV1 | CV2 | SC2 | SC3 | BASE_OFS | OFS | USR_OFS | XOFS | YOFS | G | UG | CLPS | CLP3 | CLP2 | CLP1 | CLP0 | CLPX | CLP9 | CLPS_OFS | CLP3_OFS | CLP2_OFS | CLP1_OFS | CLP0_OFS | CLPX_OFS | CLP9_OFS | aSC1A | aSC1B | aSC1C | aSC1D | aSC1E | aSC1F | aSC1G | aSC1H | aSC1I | aSC1J | aSC1K | aSC1L | aSC1M | aSC1N | aSC1O | aSC1P | SC1Q | SC1R | SC1S | SC1T | SC1U | SC1V | SC1W | SC1X | SC1Y | SC1Z | SC1AA | SC1AB | SC1AC | SC1AD | SC1AE | SC1AF | aRA | aRB | aRC | aRD | aRE | aRF | aRG | aRH | aRI | aRJ | aRK | aRL | aRM | aRN | aRO | aRP | RQ | RR | RS | RT | RU | RV | RW | RX | RY | RZ | RAA | RAB | RAC | RAD | RAE | RAF
      mask Callback dest_reg3: mbd_s32k_edma_reg_update_cbk('dest','3')
      mask Callback dest_reg3enable: mbd_s32k_edma_new_dest_reg_cbk(3)
      mask TypeOptions dest_periph4: ADC0 | ADC1 | AIPS | CAN0 | CAN1 | CAN2 | CMP0 | CRC | CSE_PRAM | DMA | DMAMUX | EIM | ENET | ERM | EWM | FLEXIO | FTFC | FTM0 | FTM1 | FTM2 | FTM3 | FTM4 | FTM5 | FTM6 | FTM7 | LMEM | LPI2C0 | LPI2C1 | LPIT0 | LPSPI0 | LPSPI1 | LPSPI2 | LPTMR0 | LPUART0 | LPUART1 | LPUART2 | MCM | MPU | MSCM | PCC | PDB0 | PDB1 | PMC | PORTA | PORTB | PORTC | PORTD | PORTE | PTA | PTB | PTC | PTD | PTE | Qu | RCM | RTC | S32_NVIC | S32_SCB | S32_SysTick | SAI0 | SAI1 | SCG | SIM | SMC | TRGMUX | WDOG
      mask Callback dest_periph4: mbd_s32k_edma_periph_update_cbk('read','dest','4')
      mask TypeOptions dest_reg4: SC1A | SC1B | SC1C | SC1D | SC1E | SC1F | SC1G | SC1H | SC1I | SC1J | SC1K | SC1L | SC1M | SC1N | SC1O | SC1P | CFG1 | CFG2 | RA | RB | RC | RD | RE | RF | RG | RH | RI | RJ | RK | RL | RM | RN | RO | RP | CV1 | CV2 | SC2 | SC3 | BASE_OFS | OFS | USR_OFS | XOFS | YOFS | G | UG | CLPS | CLP3 | CLP2 | CLP1 | CLP0 | CLPX | CLP9 | CLPS_OFS | CLP3_OFS | CLP2_OFS | CLP1_OFS | CLP0_OFS | CLPX_OFS | CLP9_OFS | aSC1A | aSC1B | aSC1C | aSC1D | aSC1E | aSC1F | aSC1G | aSC1H | aSC1I | aSC1J | aSC1K | aSC1L | aSC1M | aSC1N | aSC1O | aSC1P | SC1Q | SC1R | SC1S | SC1T | SC1U | SC1V | SC1W | SC1X | SC1Y | SC1Z | SC1AA | SC1AB | SC1AC | SC1AD | SC1AE | SC1AF | aRA | aRB | aRC | aRD | aRE | aRF | aRG | aRH | aRI | aRJ | aRK | aRL | aRM | aRN | aRO | aRP | RQ | RR | RS | RT | RU | RV | RW | RX | RY | RZ | RAA | RAB | RAC | RAD | RAE | RAF
      mask Callback dest_reg4: mbd_s32k_edma_reg_update_cbk('dest','4')
      mask Callback dest_reg4enable: mbd_s32k_edma_new_dest_reg_cbk(4)
      mask TypeOptions dest_periph5: ADC0 | ADC1 | AIPS | CAN0 | CAN1 | CAN2 | CMP0 | CRC | CSE_PRAM | DMA | DMAMUX | EIM | ENET | ERM | EWM | FLEXIO | FTFC | FTM0 | FTM1 | FTM2 | FTM3 | FTM4 | FTM5 | FTM6 | FTM7 | LMEM | LPI2C0 | LPI2C1 | LPIT0 | LPSPI0 | LPSPI1 | LPSPI2 | LPTMR0 | LPUART0 | LPUART1 | LPUART2 | MCM | MPU | MSCM | PCC | PDB0 | PDB1 | PMC | PORTA | PORTB | PORTC | PORTD | PORTE | PTA | PTB | PTC | PTD | PTE | Qu | RCM | RTC | S32_NVIC | S32_SCB | S32_SysTick | SAI0 | SAI1 | SCG | SIM | SMC | TRGMUX | WDOG
      mask Callback dest_periph5: mbd_s32k_edma_periph_update_cbk('read','dest','5')
      mask TypeOptions dest_reg5: SC1A | SC1B | SC1C | SC1D | SC1E | SC1F | SC1G | SC1H | SC1I | SC1J | SC1K | SC1L | SC1M | SC1N | SC1O | SC1P | CFG1 | CFG2 | RA | RB | RC | RD | RE | RF | RG | RH | RI | RJ | RK | RL | RM | RN | RO | RP | CV1 | CV2 | SC2 | SC3 | BASE_OFS | OFS | USR_OFS | XOFS | YOFS | G | UG | CLPS | CLP3 | CLP2 | CLP1 | CLP0 | CLPX | CLP9 | CLPS_OFS | CLP3_OFS | CLP2_OFS | CLP1_OFS | CLP0_OFS | CLPX_OFS | CLP9_OFS | aSC1A | aSC1B | aSC1C | aSC1D | aSC1E | aSC1F | aSC1G | aSC1H | aSC1I | aSC1J | aSC1K | aSC1L | aSC1M | aSC1N | aSC1O | aSC1P | SC1Q | SC1R | SC1S | SC1T | SC1U | SC1V | SC1W | SC1X | SC1Y | SC1Z | SC1AA | SC1AB | SC1AC | SC1AD | SC1AE | SC1AF | aRA | aRB | aRC | aRD | aRE | aRF | aRG | aRH | aRI | aRJ | aRK | aRL | aRM | aRN | aRO | aRP | RQ | RR | RS | RT | RU | RV | RW | RX | RY | RZ | RAA | RAB | RAC | RAD | RAE | RAF
      mask Callback dest_reg5: mbd_s32k_edma_reg_update_cbk('dest','5')
      mask Callback dest_reg5enable: mbd_s32k_edma_new_dest_reg_cbk(5)
      mask TypeOptions dest_periph6: ADC0 | ADC1 | AIPS | CAN0 | CAN1 | CAN2 | CMP0 | CRC | CSE_PRAM | DMA | DMAMUX | EIM | ENET | ERM | EWM | FLEXIO | FTFC | FTM0 | FTM1 | FTM2 | FTM3 | FTM4 | FTM5 | FTM6 | FTM7 | LMEM | LPI2C0 | LPI2C1 | LPIT0 | LPSPI0 | LPSPI1 | LPSPI2 | LPTMR0 | LPUART0 | LPUART1 | LPUART2 | MCM | MPU | MSCM | PCC | PDB0 | PDB1 | PMC | PORTA | PORTB | PORTC | PORTD | PORTE | PTA | PTB | PTC | PTD | PTE | Qu | RCM | RTC | S32_NVIC | S32_SCB | S32_SysTick | SAI0 | SAI1 | SCG | SIM | SMC | TRGMUX | WDOG
      mask Callback dest_periph6: mbd_s32k_edma_periph_update_cbk('read','dest','6')
      mask TypeOptions dest_reg6: SC1A | SC1B | SC1C | SC1D | SC1E | SC1F | SC1G | SC1H | SC1I | SC1J | SC1K | SC1L | SC1M | SC1N | SC1O | SC1P | CFG1 | CFG2 | RA | RB | RC | RD | RE | RF | RG | RH | RI | RJ | RK | RL | RM | RN | RO | RP | CV1 | CV2 | SC2 | SC3 | BASE_OFS | OFS | USR_OFS | XOFS | YOFS | G | UG | CLPS | CLP3 | CLP2 | CLP1 | CLP0 | CLPX | CLP9 | CLPS_OFS | CLP3_OFS | CLP2_OFS | CLP1_OFS | CLP0_OFS | CLPX_OFS | CLP9_OFS | aSC1A | aSC1B | aSC1C | aSC1D | aSC1E | aSC1F | aSC1G | aSC1H | aSC1I | aSC1J | aSC1K | aSC1L | aSC1M | aSC1N | aSC1O | aSC1P | SC1Q | SC1R | SC1S | SC1T | SC1U | SC1V | SC1W | SC1X | SC1Y | SC1Z | SC1AA | SC1AB | SC1AC | SC1AD | SC1AE | SC1AF | aRA | aRB | aRC | aRD | aRE | aRF | aRG | aRH | aRI | aRJ | aRK | aRL | aRM | aRN | aRO | aRP | RQ | RR | RS | RT | RU | RV | RW | RX | RY | RZ | RAA | RAB | RAC | RAD | RAE | RAF
      mask Callback dest_reg6: mbd_s32k_edma_reg_update_cbk('dest','6')
      mask Callback dest_reg6enable: mbd_s32k_edma_new_dest_reg_cbk(6)
      mask TypeOptions dest_periph7: ADC0 | ADC1 | AIPS | CAN0 | CAN1 | CAN2 | CMP0 | CRC | CSE_PRAM | DMA | DMAMUX | EIM | ENET | ERM | EWM | FLEXIO | FTFC | FTM0 | FTM1 | FTM2 | FTM3 | FTM4 | FTM5 | FTM6 | FTM7 | LMEM | LPI2C0 | LPI2C1 | LPIT0 | LPSPI0 | LPSPI1 | LPSPI2 | LPTMR0 | LPUART0 | LPUART1 | LPUART2 | MCM | MPU | MSCM | PCC | PDB0 | PDB1 | PMC | PORTA | PORTB | PORTC | PORTD | PORTE | PTA | PTB | PTC | PTD | PTE | Qu | RCM | RTC | S32_NVIC | S32_SCB | S32_SysTick | SAI0 | SAI1 | SCG | SIM | SMC | TRGMUX | WDOG
      mask Callback dest_periph7: mbd_s32k_edma_periph_update_cbk('read','dest','7')
      mask TypeOptions dest_reg7: SC1A | SC1B | SC1C | SC1D | SC1E | SC1F | SC1G | SC1H | SC1I | SC1J | SC1K | SC1L | SC1M | SC1N | SC1O | SC1P | CFG1 | CFG2 | RA | RB | RC | RD | RE | RF | RG | RH | RI | RJ | RK | RL | RM | RN | RO | RP | CV1 | CV2 | SC2 | SC3 | BASE_OFS | OFS | USR_OFS | XOFS | YOFS | G | UG | CLPS | CLP3 | CLP2 | CLP1 | CLP0 | CLPX | CLP9 | CLPS_OFS | CLP3_OFS | CLP2_OFS | CLP1_OFS | CLP0_OFS | CLPX_OFS | CLP9_OFS | aSC1A | aSC1B | aSC1C | aSC1D | aSC1E | aSC1F | aSC1G | aSC1H | aSC1I | aSC1J | aSC1K | aSC1L | aSC1M | aSC1N | aSC1O | aSC1P | SC1Q | SC1R | SC1S | SC1T | SC1U | SC1V | SC1W | SC1X | SC1Y | SC1Z | SC1AA | SC1AB | SC1AC | SC1AD | SC1AE | SC1AF | aRA | aRB | aRC | aRD | aRE | aRF | aRG | aRH | aRI | aRJ | aRK | aRL | aRM | aRN | aRO | aRP | RQ | RR | RS | RT | RU | RV | RW | RX | RY | RZ | RAA | RAB | RAC | RAD | RAE | RAF
      mask Callback dest_reg7: mbd_s32k_edma_reg_update_cbk('dest','7')
      mask Callback dest_reg7enable: mbd_s32k_edma_new_dest_reg_cbk(7)
      mask TypeOptions dest_periph8: ADC0 | ADC1 | AIPS | CAN0 | CAN1 | CAN2 | CMP0 | CRC | CSE_PRAM | DMA | DMAMUX | EIM | ENET | ERM | EWM | FLEXIO | FTFC | FTM0 | FTM1 | FTM2 | FTM3 | FTM4 | FTM5 | FTM6 | FTM7 | LMEM | LPI2C0 | LPI2C1 | LPIT0 | LPSPI0 | LPSPI1 | LPSPI2 | LPTMR0 | LPUART0 | LPUART1 | LPUART2 | MCM | MPU | MSCM | PCC | PDB0 | PDB1 | PMC | PORTA | PORTB | PORTC | PORTD | PORTE | PTA | PTB | PTC | PTD | PTE | Qu | RCM | RTC | S32_NVIC | S32_SCB | S32_SysTick | SAI0 | SAI1 | SCG | SIM | SMC | TRGMUX | WDOG
      mask Callback dest_periph8: mbd_s32k_edma_periph_update_cbk('read','dest','8')
      mask TypeOptions dest_reg8: SC1A | SC1B | SC1C | SC1D | SC1E | SC1F | SC1G | SC1H | SC1I | SC1J | SC1K | SC1L | SC1M | SC1N | SC1O | SC1P | CFG1 | CFG2 | RA | RB | RC | RD | RE | RF | RG | RH | RI | RJ | RK | RL | RM | RN | RO | RP | CV1 | CV2 | SC2 | SC3 | BASE_OFS | OFS | USR_OFS | XOFS | YOFS | G | UG | CLPS | CLP3 | CLP2 | CLP1 | CLP0 | CLPX | CLP9 | CLPS_OFS | CLP3_OFS | CLP2_OFS | CLP1_OFS | CLP0_OFS | CLPX_OFS | CLP9_OFS | aSC1A | aSC1B | aSC1C | aSC1D | aSC1E | aSC1F | aSC1G | aSC1H | aSC1I | aSC1J | aSC1K | aSC1L | aSC1M | aSC1N | aSC1O | aSC1P | SC1Q | SC1R | SC1S | SC1T | SC1U | SC1V | SC1W | SC1X | SC1Y | SC1Z | SC1AA | SC1AB | SC1AC | SC1AD | SC1AE | SC1AF | aRA | aRB | aRC | aRD | aRE | aRF | aRG | aRH | aRI | aRJ | aRK | aRL | aRM | aRN | aRO | aRP | RQ | RR | RS | RT | RU | RV | RW | RX | RY | RZ | RAA | RAB | RAC | RAD | RAE | RAF
      mask Callback dest_reg8: mbd_s32k_edma_reg_update_cbk('dest','8')
      mask Callback dest_reg8enable: mbd_s32k_edma_new_dest_reg_cbk(8)
      mask Display:
      | image('nxp_logo.png', 'top-right');
      | transfer_mode = get_param(gcb, 'transfer_mode');
      |     switch(transfer_mode)
      |         case 'Single Block Transfer'
      |             port_label('input',1,'Src address');
      |             port_label('input',2,'Dest address');
      |             port_label('input',3,'Buffer size');
      |         case 'Scatter-Gather Transfer'
      |     end
      |     port_label('output',1,'Trigger');
      | disp(maskStr);
